simulink model "debug_conversion_debug"  (R2018b)
settings: configuration reference "Active" (kept outside this file)
settings Model: DataDictionary=mloc_debug_signal_conversion.sldd  Creator=ge34qer  LastModifiedBy=ge34qer

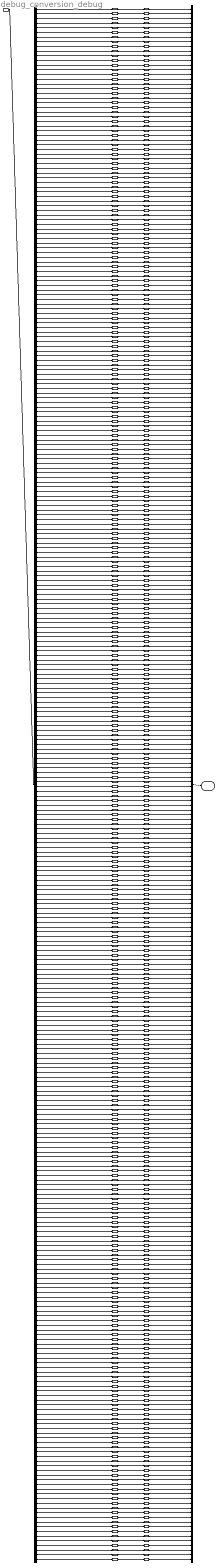
== system debug_conversion_debug ==
  debugIn : Inport  OutDataTypeStr=Bus: mvdc_vehicle_dynamics_control_debug
  BusOutput : BusSelector  OutputSignals=ErrorCode,mvdc_path_feedback_debug.Lat_FB_Sum_KappaReq_radpm,mvdc_path_feedback_debug.Lat_FB_Position,mvdc_path_feedback_debug.Lat_FB_Heading,mvdc_path_feedback_debug.Lat_LatPosError_m,mvdc_path_feedback_debug.Lat_LatPosError_DerAna_mps,mvdc_path_feedback_debug.Lat_LatPosError_DerNum_mps,mvdc_path_feedback_debug.Lat_LatPosError_DerDer_mps2,mvdc_path_feedback_debug.Lat_LatPosError_DerDerAna_mps2,mvdc_path_feedback_debug.Lat_LatPosError_DerDerNum_mps2,mvdc_path_feedback_debug.Lat_all_KappaReq_radpm,mvdc_path_matching_debug.PerformanceTrajOK_b,mvdc_path_matching_debug.EmergencyTrajOK_b,mvdc_path_matching_debug.PathPos.s_m,mvdc_path_matching_debug.PathPos.d_m,mvdc_path_matching_debug.PathPos.psi_rad,mvdc_path_matching_debug.ActualTrajPoint.LapCnt,mvdc_path_matching_debug.ActualTrajPoint.TrajCnt,mvdc_path_matching_debug.ActualTrajPoint.PointIdx,mvdc_path_matching_debug.ActualTrajPoint.s_loc_m,mvdc_path_matching_debug.ActualTrajPoint.s_glob_m,mvdc_path_matching_debug.ActualTrajPoint.x_m,mvdc_path_matching_debug.ActualTrajPoint.y_m,mvdc_path_matching_debug.ActualTrajPoint.psi_rad,mvdc_path_matching_debug.ActualTrajPoint.kappa_radpm,mvdc_path_matching_debug.ActualTrajPoint.v_mps,mvdc_path_matching_debug.ActualTrajPoint.ax_mps2,mvdc_path_matching_debug.ActualTrajPoint.banking_rad,mvdc_path_matching_debug.ActualTrajPoint.ax_lim_mps2,mvdc_path_matching_debug.ActualTrajPoint.ay_lim_mps2,mvdc_path_matching_debug.ActualTrajPoint.tube_r_m,mvdc_path_matching_debug.ActualTrajPoint.tube_l_m,mvdc_trajectory_driver_debug.ParkBrakeActive,mvdc_trajectory_driver_debug.DriverStatus,mvdc_trajectory_driver_debug.EnablePathMatching,mvdc_trajectory_driver_debug.EnableDriving,mvdc_trajectory_driver_debug.ControllerStatus,mvdc_trajectory_driver_debug.PathMatchingStatus,mvdc_trajectory_driver_debug.Strategy_Status,mvdc_trajectory_driver_debug.Trajectories_CommsStatus,mvdc_trajectory_driver_debug.Strategy_CommsStatus,mvdc_trajectory_driver_debug.tmpc_cnt,mvdc_trajectory_driver_perf.LapTime_s,mvdc_trajectory_driver_perf.e_lateral_m,mvdc_trajectory_driver_perf.eRMS_lateral_m,mvdc_trajectory_driver_perf.ePeak_lateral_m,mvdc_trajectory_driver_perf.e_heading_rad,mvdc_trajectory_driver_perf.eRMS_heading_rad,mvdc_trajectory_driver_perf.ePeak_heading_rad,mvdc_trajectory_driver_perf.e_v_mps,mvdc_trajectory_driver_perf.eRMS_v_mps,mvdc_trajectory_driver_perf.ePeak_v_mps,mvdc_trajectory_driver_perf.e_kappa_radpm,mvdc_trajectory_driver_perf.eRMS_kappa_radpm,mvdc_trajectory_driver_perf.ePeak_kappa_radpm,mvdc_trajectory_driver_perf.LongJerk_dax_mps3,mvdc_trajectory_driver_perf.LongJerkPeak_dax_mps3,mvdc_trajectory_driver_perf.LongJerkRMS_dax_mps3,mvdc_trajectory_driver_perf.LatJerk_day_mps3,mvdc_trajectory_driver_perf.LatJerkPeak_day_mps3,mvdc_trajectory_driver_perf.LatJerkRMS_day_mps3,mvdc_trajectory_driver_perf.SteeringRate_dDelta_radps,mvdc_trajectory_driver_perf.SteeringRatePeak_dDelta_radps,mvdc_trajectory_driver_perf.SteeringRateRMS_dDelta_radps,mvdc_trajectory_driver_perf.ForceRate_dF_Nps,mvdc_trajectory_driver_perf.ForceRatePeak_dF_Nps,mvdc_trajectory_driver_perf.ForceRateRMS_dF_Nps,mvdc_trajectory_driver_perf.LatConstViolations,mvdc_trajectory_driver_perf.TireConstViolations,mvdc_trajectory_driver_perf.TireUtilization,mvdc_trajectory_driver_perf.TireUtilization_c1,mvdc_trajectory_driver_perf.TireUtilization_c2,mvdc_curvvel_tracking_debug.Curv_TargetAy_mps2,mvdc_curvvel_tracking_debug.Curv_all_KappaReq_radpm,mvdc_curvvel_tracking_debug.Curv_FB_Dist_DeltaReq_rad,mvdc_curvvel_tracking_debug.Curv_FB_Diff_DeltaReq_rad,mvdc_curvvel_tracking_debug.Curv_FF_Kappa_DeltaReq_rad,mvdc_curvvel_tracking_debug.Curv_USComp_DeltaReq_rad,mvdc_curvvel_tracking_debug.Curv_CurvError_radpm,mvdc_curvvel_tracking_debug.Curv_TargetCurv_radpm,mvdc_curvvel_tracking_debug.Long_FB_Dist_FxReq_N,mvdc_curvvel_tracking_debug.Long_FF_Dist_FxReq_N,mvdc_curvvel_tracking_debug.Long_FB_VelDiff_FxReq_N,mvdc_curvvel_tracking_debug.Long_FF_Traj_FxReq_N,mvdc_curvvel_tracking_debug.Long_VelError_mps,mvdc_curvvel_tracking_debug.Long_TargetSpeed_mps,mvdc_curvvel_tracking_debug.Long_axTarget_mps2,mvdc_curvvel_tracking_debug.Req_Delta_rad,mvdc_curvvel_tracking_debug.Req_Fx_N,mvdc_curvvel_tracking_debug.ControlState,mvdc_curvvel_tracking_debug.EnableDriving,mvdc_curvvel_tracking_debug.EnableEmergency,mvdc_tmpc_fast_debug.LatAcc_bank_mps2,mvdc_tmpc_fast_debug.LatAcc_FB_Dist_rad,mvdc_tmpc_fast_debug.LatAcc_FB_ay_rad,mvdc_tmpc_fast_debug.LatAcc_FB_Delta_rad,mvdc_tmpc_fast_debug.LatAcc_FFss_rad,mvdc_tmpc_fast_debug.LatAcc_FFdyn_rad,mvdc_tmpc_fast_debug.LatAcc_Control_rad,mvdc_tmpc_fast_debug.LatAcc_Target_mps2,mvdc_tmpc_fast_debug.LatAcc_VirtualAccTarget_mps2,mvdc_tmpc_fast_debug.LatAcc_VirtualSteeringTarget_rad,mvdc_tmpc_fast_debug.LatAcc_FFLearned_rad,mvdc_tmpc_fast_debug.LatAcc_DiffToNeutralSteer_rad,mvdc_tmpc_fast_debug.LatAcc_FBStabilizer_rad,mvdc_tmpc_fast_debug.LongAcc_FB_N,mvdc_tmpc_fast_debug.LongAcc_FFax_N,mvdc_tmpc_fast_debug.LongAcc_FFdist_N,mvdc_tmpc_fast_debug.LongAcc_Control_N,mvdc_tmpc_fast_debug.LongAcc_Target_mps2,mvdc_tmpc_fast_debug.LongAcc_TargetFF_mps2,mvdc_tmpc_fast_debug.LongAcc_FFLearned_N,mvdc_tmpc_fast_debug.state_cost,mvdc_tmpc_fast_debug.input_cost,mvdc_tmpc_fast_debug.reg_cost,mvdc_tmpc_fast_debug.slack_cost,mvdc_tmpc_fast_debug.solver_iteration,mvdc_tmpc_fast_debug.solver_state,mvdc_tmpc_fast_debug.solver_runTime_s,mvdc_tmpc_fast_debug.solver_pri_res,mvdc_tmpc_fast_debug.solver_dua_res,mvdc_tmpc_fast_debug.tmpc_cnt,mvdc_tmpc_fast_debug.TireUtilizationTarget,mvdc_tmpc_fast_debug.ax_LearnedBound_mps2,mvdc_tmpc_fast_debug.ax_DataCoverage_perc,mvdc_tmpc_fast_debug.ax_Uncertainty_mps2,mvdc_tmpc_fast_debug.ay_LearnedBound_mps2,mvdc_tmpc_fast_debug.ay_DataCoverage_perc,mvdc_tmpc_fast_debug.ay_Uncertainty_mps2,mvdc_tmpc_fast_debug.dot_d_analytical_mps,mvdc_tmpc_fast_debug.dot_d_numerical_mps,mvdc_actuator_debug.steering_delta_target_rad,mvdc_actuator_debug.steering_delta_error_rad,mvdc_actuator_debug.steering_delta_FB_rad,mvdc_actuator_debug.steering_delta_FB_p_rad,mvdc_actuator_debug.steering_delta_FB_i_rad,mvdc_actuator_debug.steering_delta_FB_d_rad,mvdc_actuator_debug.steering_delta_FF_rad,mvdc_actuator_debug.RequestSteeringAngle_rad,mvdc_actuator_debug.RequestLongForce_N,mvdc_actuator_debug.TCCorrectiveForce_N,mvdc_actuator_debug.TCSlipDifference_perc,mvdc_actuator_debug.TCProportionalForce_N,mvdc_actuator_debug.TCIntegralForce_N,mvdc_actuator_debug.T_request_Nm,mvdc_actuator_debug.T_max_Nm,mvdc_actuator_debug.T_min_Nm,mvdc_actuator_debug.T_engine_Nm,mvdc_actuator_debug.p_Brake_bar,mvdc_actuator_debug.p_throttle_pos,mvdc_actuator_debug.gear,ExternalDebug.UnixTime_s,ExternalDebug.ExecutionTime_s,ExternalDebug.ControlTime_s,ExternalDebug.UpdateFrequency_Hz,ExternalDebug.LostHeartbeatTimeout_s,ExternalDebug.LostRaceControlTimeout_s,ExternalDebug.DiagSD,ExternalDebug.DiagMotec,ExternalDebug.DiagOther,mvdc_state_estimation_debug.StateEstimate.SE_Status,mvdc_state_estimation_debug.StateEstimate.SE_State,mvdc_state_estimation_debug.StateEstimate.Pos.x_m,mvdc_state_estimation_debug.StateEstimate.Pos.y_m,mvdc_state_estimation_debug.StateEstimate.Pos.psi_rad,mvdc_state_estimation_debug.StateEstimate.z_m,mvdc_state_estimation_debug.StateEstimate.PosAccuracy,mvdc_state_estimation_debug.StateEstimate.VelAccuracy,mvdc_state_estimation_debug.StateEstimate.dPsi_radps,mvdc_state_estimation_debug.StateEstimate.vx_mps,mvdc_state_estimation_debug.StateEstimate.vy_mps,mvdc_state_estimation_debug.StateEstimate.v_mps,mvdc_state_estimation_debug.StateEstimate.beta_rad,mvdc_state_estimation_debug.StateEstimate.ax_mps2,mvdc_state_estimation_debug.StateEstimate.ay_mps2,mvdc_state_estimation_debug.StateEstimate.valid_IMU_b,mvdc_state_estimation_debug.StateEstimate.psi_vel_rad,mvdc_state_estimation_debug.StateEstimate.kappa_radpm,mvdc_state_estimation_debug.StateEstimate.dBeta_radps,mvdc_state_estimation_debug.StateEstimate.ddPsi_radps2,mvdc_state_estimation_debug.StateEstimate.ax_vel_mps2,mvdc_state_estimation_debug.StateEstimate.ay_vel_mps2,mvdc_state_estimation_debug.StateEstimate.lambdaFL_perc,mvdc_state_estimation_debug.StateEstimate.lambdaFR_perc,mvdc_state_estimation_debug.StateEstimate.lambdaRL_perc,mvdc_state_estimation_debug.StateEstimate.lambdaRR_perc,mvdc_state_estimation_debug.StateEstimate.valid_Wheelspeeds_b,mvdc_state_estimation_debug.StateEstimate.alphaFL_rad,mvdc_state_estimation_debug.StateEstimate.alphaFR_rad,mvdc_state_estimation_debug.StateEstimate.alphaRL_rad,mvdc_state_estimation_debug.StateEstimate.alphaRR_rad,mvdc_state_estimation_debug.StateEstimate.DiffFRAlpha_rad,mvdc_state_estimation_debug.StateEstimate.DeltaWheel_rad,mvdc_state_estimation_debug.Residuals.res_xLoc1_m,mvdc_state_estimation_debug.Residuals.res_yLoc1_m,mvdc_state_estimation_debug.Residuals.res_psiLoc1_rad,mvdc_state_estimation_debug.Residuals.res_xLoc2_m,mvdc_state_estimation_debug.Residuals.res_yLoc2_m,mvdc_state_estimation_debug.Residuals.res_psiLoc2_rad,mvdc_state_estimation_debug.Residuals.res_xLoc3_m,mvdc_state_estimation_debug.Residuals.res_yLoc3_m,mvdc_state_estimation_debug.Residuals.res_psiLoc3_rad,mvdc_state_estimation_debug.Residuals.res_vxVel1_mps,mvdc_state_estimation_debug.Residuals.res_vyVel1_mps,mvdc_state_estimation_debug.Residuals.res_vxVel2_mps,mvdc_state_estimation_debug.Residuals.res_vyVel2_mps,mvdc_state_estimation_debug.Residuals.res_dPsi1_radps,mvdc_state_estimation_debug.Residuals.res_dPsi2_radps,mvdc_state_estimation_debug.Residuals.res_sLoc1_m,mvdc_state_estimation_debug.Residuals.res_dLoc1_m,mvdc_state_estimation_debug.Residuals.res_sLoc2_m,mvdc_state_estimation_debug.Residuals.res_dLoc2_m,mvdc_state_estimation_debug.Residuals.res_sLoc3_m,mvdc_state_estimation_debug.Residuals.res_dLoc3_m,mvdc_state_estimation_debug.Diagnosis.valid_Loc1_b,mvdc_state_estimation_debug.Diagnosis.valid_Loc2_b,mvdc_state_estimation_debug.Diagnosis.valid_Loc3_b,mvdc_state_estimation_debug.Diagnosis.valid_Vel1_b,mvdc_state_estimation_debug.Diagnosis.valid_Vel2_b,mvdc_state_estimation_debug.Diagnosis.valid_IMU1_b,mvdc_state_estimation_debug.Diagnosis.valid_IMU2_b,mvdc_state_estimation_debug.Diagnosis.fail_Loc1_b,mvdc_state_estimation_debug.Diagnosis.fail_Loc2_b,mvdc_state_estimation_debug.Diagnosis.fail_Loc3_b,mvdc_state_estimation_debug.Diagnosis.fail_Vel1_b,mvdc_state_estimation_debug.Diagnosis.fail_Vel2_b,mvdc_state_estimation_debug.Diagnosis.fail_IMU1_b,mvdc_state_estimation_debug.Diagnosis.fail_IMU2_b,mvdc_state_estimation_debug.Odom.Position.x_m,mvdc_state_estimation_debug.Odom.Position.y_m,mvdc_state_estimation_debug.Odom.Position.psi_rad,mvdc_state_estimation_debug.Odom.Valid_b,mloc_statemachine_debug.Hardware_Status,mloc_statemachine_debug.AIDriver_Status,mloc_statemachine_debug.ParkBrakeApplied_b,mloc_statemachine_debug.VehicleReady2Drive,mloc_statemachine_debug.StateEstimation_Status,mloc_statemachine_debug.VehicleSafeStandstill,mloc_statemachine_debug.Driver_Status,mloc_statemachine_debug.VehicleUnsafe,mloc_statemachine_debug.TUMVehicleState,mloc_statemachine_debug.EnableSensorFusion,mloc_statemachine_debug.EnableControlOutputs,mloc_statemachine_debug.EnableDriver,mloc_statemachine_debug.EnableHardEmergencyBrake,mloc_statemachine_debug.RequestControl,VehicleSensorData.s_DamperPotsFL_mm,VehicleSensorData.s_DamperPotsFR_mm,VehicleSensorData.s_DamperPotsRL_mm,VehicleSensorData.s_DamperPotsRR_mm,VehicleSensorData.p_TirePressureFL_bar,VehicleSensorData.p_TirePressureFR_bar,VehicleSensorData.p_TirePressureRL_bar,VehicleSensorData.p_TirePressureRR_bar,VehicleSensorData.T_TireFL_Celsius,VehicleSensorData.T_TireFR_Celsius,VehicleSensorData.T_TireRL_Celsius,VehicleSensorData.T_TireRR_Celsius,VehicleSensorData.BatteryVoltage_V,VehicleSensorData.Delta_Manual_rad,VehicleSensorData.Throttle_Manual_perc,VehicleSensorData.Brake_Manual_bar,VehicleSensorData.Gear_Manual,VehicleSensorData.T_CoolantTemp_Celsius,VehicleSensorData.T_TransmissionOilTemp_Celsius,VehicleSensorData.p_Fuel_kPa,VehicleSensorData.p_EngineOil_kPa,VehicleSensorData.Tz_Powertrain_Nm,VehicleSensorData.T_Engine_Nm,VehicleSensorData.GearEngaged,VehicleSensorData.omega_Engine_radps,VehicleSensorData.ThrottlePos_perc,VehicleSensorData.T_WheelFL_Nm,VehicleSensorData.T_WheelFR_Nm,VehicleSensorData.T_WheelRL_Nm,VehicleSensorData.T_WheelRR_Nm,VehicleSensorData.Delta_Wheel_rad,VehicleSensorData.p_BrakeF_bar,VehicleSensorData.p_BrakeR_bar,VehicleSensorData.omega_WheelFL_radps,VehicleSensorData.omega_WheelFR_radps,VehicleSensorData.omega_WheelRL_radps,VehicleSensorData.omega_WheelRR_radps,VehicleSensorData.valid_Wheelspeeds_b,VehicleSensorData.x_Loc1_m,VehicleSensorData.y_Loc1_m,VehicleSensorData.z_Loc1_m,VehicleSensorData.phi_RollAngleLoc1_rad,VehicleSensorData.theta_PitchAngleLoc1_rad,VehicleSensorData.psi_YawAngleLoc1_rad,VehicleSensorData.t_EstimateLoc1_s,VehicleSensorData.valid_Loc1_b,VehicleSensorData.accuracy_Loc1,VehicleSensorData.x_Loc2_m,VehicleSensorData.y_Loc2_m,VehicleSensorData.z_Loc2_m,VehicleSensorData.phi_RollAngleLoc2_rad,VehicleSensorData.theta_PitchAngleLoc2_rad,VehicleSensorData.psi_YawAngleLoc2_rad,VehicleSensorData.t_EstimateLoc2_s,VehicleSensorData.valid_Loc2_b,VehicleSensorData.accuracy_Loc2,VehicleSensorData.x_Loc3_m,VehicleSensorData.y_Loc3_m,VehicleSensorData.z_Loc3_m,VehicleSensorData.phi_RollAngleLoc3_rad,VehicleSensorData.theta_PitchAngleLoc3_rad,VehicleSensorData.psi_YawAngleLoc3_rad,VehicleSensorData.t_EstimateLoc3_s,VehicleSensorData.valid_Loc3_b,VehicleSensorData.accuracy_Loc3,VehicleSensorData.vx_CoGVel1_mps,VehicleSensorData.vy_CoGVel1_mps,VehicleSensorData.valid_Vel1_b,VehicleSensorData.vx_CoGVel2_mps,VehicleSensorData.vy_CoGVel2_mps,VehicleSensorData.valid_Vel2_b,VehicleSensorData.ax_CoGIMU1_mps2,VehicleSensorData.ay_CoGIMU1_mps2,VehicleSensorData.az_CoGIMU1_mps2,VehicleSensorData.dPhi_RollRateIMU1_radps,VehicleSensorData.dTheta_PitchRateIMU1_radps,VehicleSensorData.dPsi_YawRateIMU1_radps,VehicleSensorData.valid_IMU1_b,VehicleSensorData.ax_CoGIMU2_mps2,VehicleSensorData.ay_CoGIMU2_mps2,VehicleSensorData.az_CoGIMU2_mps2,VehicleSensorData.dPhi_RollRateIMU2_radps,VehicleSensorData.dTheta_PitchRateIMU2_radps,VehicleSensorData.dPsi_YawRateIMU2_radps,VehicleSensorData.valid_IMU2_b,Time_s
  Convert{1..332} (332 alike) : DataTypeConversion  OutDataTypeStr=double  SaturateOnIntegerOverflow=on  RndMeth=Zero
  Mux : Mux  Inputs=332
  debug_ErrorCode : SignalConversion  OverrideOpt=off
  debug_ExternalDebug_ControlTime_s : SignalConversion  OverrideOpt=off
  debug_ExternalDebug_DiagMotec : SignalConversion  OverrideOpt=off
  debug_ExternalDebug_DiagOther : SignalConversion  OverrideOpt=off
  debug_ExternalDebug_DiagSD : SignalConversion  OverrideOpt=off
  debug_ExternalDebug_ExecutionTime_s : SignalConversion  OverrideOpt=off
  debug_ExternalDebug_LostHeartbeatTimeout_s : SignalConversion  OverrideOpt=off
  debug_ExternalDebug_LostRaceControlTimeout_s : SignalConversion  OverrideOpt=off
  debug_ExternalDebug_UnixTime_s : SignalConversion  OverrideOpt=off
  debug_ExternalDebug_UpdateFrequency_Hz : SignalConversion  OverrideOpt=off
  debug_Time_s : SignalConversion  OverrideOpt=off
  debug_VehicleSensorData_BatteryVoltage_V : SignalConversion  OverrideOpt=off
  debug_VehicleSensorData_Brake_Manual_bar : SignalConversion  OverrideOpt=off
  debug_VehicleSensorData_Delta_Manual_rad : SignalConversion  OverrideOpt=off
  debug_VehicleSensorData_Delta_Wheel_rad : SignalConversion  OverrideOpt=off
  debug_VehicleSensorData_GearEngaged : SignalConversion  OverrideOpt=off
  debug_VehicleSensorData_Gear_Manual : SignalConversion  OverrideOpt=off
  debug_VehicleSensorData_T_CoolantTemp_Celsius : SignalConversion  OverrideOpt=off
  debug_VehicleSensorData_T_Engine_Nm : SignalConversion  OverrideOpt=off
  debug_VehicleSensorData_T_TireFL_Celsius : SignalConversion  OverrideOpt=off
  debug_VehicleSensorData_T_TireFR_Celsius : SignalConversion  OverrideOpt=off
  debug_VehicleSensorData_T_TireRL_Celsius : SignalConversion  OverrideOpt=off
  debug_VehicleSensorData_T_TireRR_Celsius : SignalConversion  OverrideOpt=off
  debug_VehicleSensorData_T_TransmissionOilTemp_Celsius : SignalConversion  OverrideOpt=off
  debug_VehicleSensorData_T_WheelFL_Nm : SignalConversion  OverrideOpt=off
  debug_VehicleSensorData_T_WheelFR_Nm : SignalConversion  OverrideOpt=off
  debug_VehicleSensorData_T_WheelRL_Nm : SignalConversion  OverrideOpt=off
  debug_VehicleSensorData_T_WheelRR_Nm : SignalConversion  OverrideOpt=off
  debug_VehicleSensorData_ThrottlePos_perc : SignalConversion  OverrideOpt=off
  debug_VehicleSensorData_Throttle_Manual_perc : SignalConversion  OverrideOpt=off
  debug_VehicleSensorData_Tz_Powertrain_Nm : SignalConversion  OverrideOpt=off
  debug_VehicleSensorData_accuracy_Loc1 : SignalConversion  OverrideOpt=off
  debug_VehicleSensorData_accuracy_Loc2 : SignalConversion  OverrideOpt=off
  debug_VehicleSensorData_accuracy_Loc3 : SignalConversion  OverrideOpt=off
  debug_VehicleSensorData_ax_CoGIMU1_mps2 : SignalConversion  OverrideOpt=off
  debug_VehicleSensorData_ax_CoGIMU2_mps2 : SignalConversion  OverrideOpt=off
  debug_VehicleSensorData_ay_CoGIMU1_mps2 : SignalConversion  OverrideOpt=off
  debug_VehicleSensorData_ay_CoGIMU2_mps2 : SignalConversion  OverrideOpt=off
  debug_VehicleSensorData_az_CoGIMU1_mps2 : SignalConversion  OverrideOpt=off
  debug_VehicleSensorData_az_CoGIMU2_mps2 : SignalConversion  OverrideOpt=off
  debug_VehicleSensorData_dPhi_RollRateIMU1_radps : SignalConversion  OverrideOpt=off
  debug_VehicleSensorData_dPhi_RollRateIMU2_radps : SignalConversion  OverrideOpt=off
  debug_VehicleSensorData_dPsi_YawRateIMU1_radps : SignalConversion  OverrideOpt=off
  debug_VehicleSensorData_dPsi_YawRateIMU2_radps : SignalConversion  OverrideOpt=off
  debug_VehicleSensorData_dTheta_PitchRateIMU1_radps : SignalConversion  OverrideOpt=off
  debug_VehicleSensorData_dTheta_PitchRateIMU2_radps : SignalConversion  OverrideOpt=off
  debug_VehicleSensorData_omega_Engine_radps : SignalConversion  OverrideOpt=off
  debug_VehicleSensorData_omega_WheelFL_radps : SignalConversion  OverrideOpt=off
  debug_VehicleSensorData_omega_WheelFR_radps : SignalConversion  OverrideOpt=off
  debug_VehicleSensorData_omega_WheelRL_radps : SignalConversion  OverrideOpt=off
  debug_VehicleSensorData_omega_WheelRR_radps : SignalConversion  OverrideOpt=off
  debug_VehicleSensorData_p_BrakeF_bar : SignalConversion  OverrideOpt=off
  debug_VehicleSensorData_p_BrakeR_bar : SignalConversion  OverrideOpt=off
  debug_VehicleSensorData_p_EngineOil_kPa : SignalConversion  OverrideOpt=off
  debug_VehicleSensorData_p_Fuel_kPa : SignalConversion  OverrideOpt=off
  debug_VehicleSensorData_p_TirePressureFL_bar : SignalConversion  OverrideOpt=off
  debug_VehicleSensorData_p_TirePressureFR_bar : SignalConversion  OverrideOpt=off
  debug_VehicleSensorData_p_TirePressureRL_bar : SignalConversion  OverrideOpt=off
  debug_VehicleSensorData_p_TirePressureRR_bar : SignalConversion  OverrideOpt=off
  debug_VehicleSensorData_phi_RollAngleLoc1_rad : SignalConversion  OverrideOpt=off
  debug_VehicleSensorData_phi_RollAngleLoc2_rad : SignalConversion  OverrideOpt=off
  debug_VehicleSensorData_phi_RollAngleLoc3_rad : SignalConversion  OverrideOpt=off
  debug_VehicleSensorData_psi_YawAngleLoc1_rad : SignalConversion  OverrideOpt=off
  debug_VehicleSensorData_psi_YawAngleLoc2_rad : SignalConversion  OverrideOpt=off
  debug_VehicleSensorData_psi_YawAngleLoc3_rad : SignalConversion  OverrideOpt=off
  debug_VehicleSensorData_s_DamperPotsFL_mm : SignalConversion  OverrideOpt=off
  debug_VehicleSensorData_s_DamperPotsFR_mm : SignalConversion  OverrideOpt=off
  debug_VehicleSensorData_s_DamperPotsRL_mm : SignalConversion  OverrideOpt=off
  debug_VehicleSensorData_s_DamperPotsRR_mm : SignalConversion  OverrideOpt=off
  debug_VehicleSensorData_t_EstimateLoc1_s : SignalConversion  OverrideOpt=off
  debug_VehicleSensorData_t_EstimateLoc2_s : SignalConversion  OverrideOpt=off
  debug_VehicleSensorData_t_EstimateLoc3_s : SignalConversion  OverrideOpt=off
  debug_VehicleSensorData_theta_PitchAngleLoc1_rad : SignalConversion  OverrideOpt=off
  debug_VehicleSensorData_theta_PitchAngleLoc2_rad : SignalConversion  OverrideOpt=off
  debug_VehicleSensorData_theta_PitchAngleLoc3_rad : SignalConversion  OverrideOpt=off
  debug_VehicleSensorData_valid_IMU1_b : SignalConversion  OverrideOpt=off
  debug_VehicleSensorData_valid_IMU2_b : SignalConversion  OverrideOpt=off
  debug_VehicleSensorData_valid_Loc1_b : SignalConversion  OverrideOpt=off
  debug_VehicleSensorData_valid_Loc2_b : SignalConversion  OverrideOpt=off
  debug_VehicleSensorData_valid_Loc3_b : SignalConversion  OverrideOpt=off
  debug_VehicleSensorData_valid_Vel1_b : SignalConversion  OverrideOpt=off
  debug_VehicleSensorData_valid_Vel2_b : SignalConversion  OverrideOpt=off
  debug_VehicleSensorData_valid_Wheelspeeds_b : SignalConversion  OverrideOpt=off
  debug_VehicleSensorData_vx_CoGVel1_mps : SignalConversion  OverrideOpt=off
  debug_VehicleSensorData_vx_CoGVel2_mps : SignalConversion  OverrideOpt=off
  debug_VehicleSensorData_vy_CoGVel1_mps : SignalConversion  OverrideOpt=off
  debug_VehicleSensorData_vy_CoGVel2_mps : SignalConversion  OverrideOpt=off
  debug_VehicleSensorData_x_Loc1_m : SignalConversion  OverrideOpt=off
  debug_VehicleSensorData_x_Loc2_m : SignalConversion  OverrideOpt=off
  debug_VehicleSensorData_x_Loc3_m : SignalConversion  OverrideOpt=off
  debug_VehicleSensorData_y_Loc1_m : SignalConversion  OverrideOpt=off
  debug_VehicleSensorData_y_Loc2_m : SignalConversion  OverrideOpt=off
  debug_VehicleSensorData_y_Loc3_m : SignalConversion  OverrideOpt=off
  debug_VehicleSensorData_z_Loc1_m : SignalConversion  OverrideOpt=off
  debug_VehicleSensorData_z_Loc2_m : SignalConversion  OverrideOpt=off
  debug_VehicleSensorData_z_Loc3_m : SignalConversion  OverrideOpt=off
  debug_mloc_statemachine_debug_AIDriver_Status : SignalConversion  OverrideOpt=off
  debug_mloc_statemachine_debug_Driver_Status : SignalConversion  OverrideOpt=off
  debug_mloc_statemachine_debug_EnableControlOutputs : SignalConversion  OverrideOpt=off
  debug_mloc_statemachine_debug_EnableDriver : SignalConversion  OverrideOpt=off
  debug_mloc_statemachine_debug_EnableHardEmergencyBrake : SignalConversion  OverrideOpt=off
  debug_mloc_statemachine_debug_EnableSensorFusion : SignalConversion  OverrideOpt=off
  debug_mloc_statemachine_debug_Hardware_Status : SignalConversion  OverrideOpt=off
  debug_mloc_statemachine_debug_ParkBrakeApplied_b : SignalConversion  OverrideOpt=off
  debug_mloc_statemachine_debug_RequestControl : SignalConversion  OverrideOpt=off
  debug_mloc_statemachine_debug_StateEstimation_Status : SignalConversion  OverrideOpt=off
  debug_mloc_statemachine_debug_TUMVehicleState : SignalConversion  OverrideOpt=off
  debug_mloc_statemachine_debug_VehicleReady2Drive : SignalConversion  OverrideOpt=off
  debug_mloc_statemachine_debug_VehicleSafeStandstill : SignalConversion  OverrideOpt=off
  debug_mloc_statemachine_debug_VehicleUnsafe : SignalConversion  OverrideOpt=off
  debug_mvdc_actuator_debug_RequestLongForce_N : SignalConversion  OverrideOpt=off
  debug_mvdc_actuator_debug_RequestSteeringAngle_rad : SignalConversion  OverrideOpt=off
  debug_mvdc_actuator_debug_TCCorrectiveForce_N : SignalConversion  OverrideOpt=off
  debug_mvdc_actuator_debug_TCIntegralForce_N : SignalConversion  OverrideOpt=off
  debug_mvdc_actuator_debug_TCProportionalForce_N : SignalConversion  OverrideOpt=off
  debug_mvdc_actuator_debug_TCSlipDifference_perc : SignalConversion  OverrideOpt=off
  debug_mvdc_actuator_debug_T_engine_Nm : SignalConversion  OverrideOpt=off
  debug_mvdc_actuator_debug_T_max_Nm : SignalConversion  OverrideOpt=off
  debug_mvdc_actuator_debug_T_min_Nm : SignalConversion  OverrideOpt=off
  debug_mvdc_actuator_debug_T_request_Nm : SignalConversion  OverrideOpt=off
  debug_mvdc_actuator_debug_gear : SignalConversion  OverrideOpt=off
  debug_mvdc_actuator_debug_p_Brake_bar : SignalConversion  OverrideOpt=off
  debug_mvdc_actuator_debug_p_throttle_pos : SignalConversion  OverrideOpt=off
  debug_mvdc_actuator_debug_steering_delta_FB_d_rad : SignalConversion  OverrideOpt=off
  debug_mvdc_actuator_debug_steering_delta_FB_i_rad : SignalConversion  OverrideOpt=off
  debug_mvdc_actuator_debug_steering_delta_FB_p_rad : SignalConversion  OverrideOpt=off
  debug_mvdc_actuator_debug_steering_delta_FB_rad : SignalConversion  OverrideOpt=off
  debug_mvdc_actuator_debug_steering_delta_FF_rad : SignalConversion  OverrideOpt=off
  debug_mvdc_actuator_debug_steering_delta_error_rad : SignalConversion  OverrideOpt=off
  debug_mvdc_actuator_debug_steering_delta_target_rad : SignalConversion  OverrideOpt=off
  debug_mvdc_curvvel_tracking_debug_ControlState : SignalConversion  OverrideOpt=off
  debug_mvdc_curvvel_tracking_debug_Curv_CurvError_radpm : SignalConversion  OverrideOpt=off
  debug_mvdc_curvvel_tracking_debug_Curv_FB_Diff_DeltaReq_rad : SignalConversion  OverrideOpt=off
  debug_mvdc_curvvel_tracking_debug_Curv_FB_Dist_DeltaReq_rad : SignalConversion  OverrideOpt=off
  debug_mvdc_curvvel_tracking_debug_Curv_FF_Kappa_DeltaReq_rad : SignalConversion  OverrideOpt=off
  debug_mvdc_curvvel_tracking_debug_Curv_TargetAy_mps2 : SignalConversion  OverrideOpt=off
  debug_mvdc_curvvel_tracking_debug_Curv_TargetCurv_radpm : SignalConversion  OverrideOpt=off
  debug_mvdc_curvvel_tracking_debug_Curv_USComp_DeltaReq_rad : SignalConversion  OverrideOpt=off
  debug_mvdc_curvvel_tracking_debug_Curv_all_KappaReq_radpm : SignalConversion  OverrideOpt=off
  debug_mvdc_curvvel_tracking_debug_EnableDriving : SignalConversion  OverrideOpt=off
  debug_mvdc_curvvel_tracking_debug_EnableEmergency : SignalConversion  OverrideOpt=off
  debug_mvdc_curvvel_tracking_debug_Long_FB_Dist_FxReq_N : SignalConversion  OverrideOpt=off
  debug_mvdc_curvvel_tracking_debug_Long_FB_VelDiff_FxReq_N : SignalConversion  OverrideOpt=off
  debug_mvdc_curvvel_tracking_debug_Long_FF_Dist_FxReq_N : SignalConversion  OverrideOpt=off
  debug_mvdc_curvvel_tracking_debug_Long_FF_Traj_FxReq_N : SignalConversion  OverrideOpt=off
  debug_mvdc_curvvel_tracking_debug_Long_TargetSpeed_mps : SignalConversion  OverrideOpt=off
  debug_mvdc_curvvel_tracking_debug_Long_VelError_mps : SignalConversion  OverrideOpt=off
  debug_mvdc_curvvel_tracking_debug_Long_axTarget_mps2 : SignalConversion  OverrideOpt=off
  debug_mvdc_curvvel_tracking_debug_Req_Delta_rad : SignalConversion  OverrideOpt=off
  debug_mvdc_curvvel_tracking_debug_Req_Fx_N : SignalConversion  OverrideOpt=off
  debug_mvdc_path_feedback_debug_Lat_FB_Heading : SignalConversion  OverrideOpt=off
  debug_mvdc_path_feedback_debug_Lat_FB_Position : SignalConversion  OverrideOpt=off
  debug_mvdc_path_feedback_debug_Lat_FB_Sum_KappaReq_radpm : SignalConversion  OverrideOpt=off
  debug_mvdc_path_feedback_debug_Lat_LatPosError_DerAna_mps : SignalConversion  OverrideOpt=off
  debug_mvdc_path_feedback_debug_Lat_LatPosError_DerDerAna_mps2 : SignalConversion  OverrideOpt=off
  debug_mvdc_path_feedback_debug_Lat_LatPosError_DerDerNum_mps2 : SignalConversion  OverrideOpt=off
  debug_mvdc_path_feedback_debug_Lat_LatPosError_DerDer_mps2 : SignalConversion  OverrideOpt=off
  debug_mvdc_path_feedback_debug_Lat_LatPosError_DerNum_mps : SignalConversion  OverrideOpt=off
  debug_mvdc_path_feedback_debug_Lat_LatPosError_m : SignalConversion  OverrideOpt=off
  debug_mvdc_path_feedback_debug_Lat_all_KappaReq_radpm : SignalConversion  OverrideOpt=off
  debug_mvdc_path_matching_debug_ActualTrajPoint_LapCnt : SignalConversion  OverrideOpt=off
  debug_mvdc_path_matching_debug_ActualTrajPoint_PointIdx : SignalConversion  OverrideOpt=off
  debug_mvdc_path_matching_debug_ActualTrajPoint_TrajCnt : SignalConversion  OverrideOpt=off
  debug_mvdc_path_matching_debug_ActualTrajPoint_ax_lim_mps2 : SignalConversion  OverrideOpt=off
  debug_mvdc_path_matching_debug_ActualTrajPoint_ax_mps2 : SignalConversion  OverrideOpt=off
  debug_mvdc_path_matching_debug_ActualTrajPoint_ay_lim_mps2 : SignalConversion  OverrideOpt=off
  debug_mvdc_path_matching_debug_ActualTrajPoint_banking_rad : SignalConversion  OverrideOpt=off
  debug_mvdc_path_matching_debug_ActualTrajPoint_kappa_radpm : SignalConversion  OverrideOpt=off
  debug_mvdc_path_matching_debug_ActualTrajPoint_psi_rad : SignalConversion  OverrideOpt=off
  debug_mvdc_path_matching_debug_ActualTrajPoint_s_glob_m : SignalConversion  OverrideOpt=off
  debug_mvdc_path_matching_debug_ActualTrajPoint_s_loc_m : SignalConversion  OverrideOpt=off
  debug_mvdc_path_matching_debug_ActualTrajPoint_tube_l_m : SignalConversion  OverrideOpt=off
  debug_mvdc_path_matching_debug_ActualTrajPoint_tube_r_m : SignalConversion  OverrideOpt=off
  debug_mvdc_path_matching_debug_ActualTrajPoint_v_mps : SignalConversion  OverrideOpt=off
  debug_mvdc_path_matching_debug_ActualTrajPoint_x_m : SignalConversion  OverrideOpt=off
  debug_mvdc_path_matching_debug_ActualTrajPoint_y_m : SignalConversion  OverrideOpt=off
  debug_mvdc_path_matching_debug_EmergencyTrajOK_b : SignalConversion  OverrideOpt=off
  debug_mvdc_path_matching_debug_PathPos_d_m : SignalConversion  OverrideOpt=off
  debug_mvdc_path_matching_debug_PathPos_psi_rad : SignalConversion  OverrideOpt=off
  debug_mvdc_path_matching_debug_PathPos_s_m : SignalConversion  OverrideOpt=off
  debug_mvdc_path_matching_debug_PerformanceTrajOK_b : SignalConversion  OverrideOpt=off
  debug_mvdc_state_estimation_debug_Diagnosis_fail_IMU1_b : SignalConversion  OverrideOpt=off
  debug_mvdc_state_estimation_debug_Diagnosis_fail_IMU2_b : SignalConversion  OverrideOpt=off
  debug_mvdc_state_estimation_debug_Diagnosis_fail_Loc1_b : SignalConversion  OverrideOpt=off
  debug_mvdc_state_estimation_debug_Diagnosis_fail_Loc2_b : SignalConversion  OverrideOpt=off
  debug_mvdc_state_estimation_debug_Diagnosis_fail_Loc3_b : SignalConversion  OverrideOpt=off
  debug_mvdc_state_estimation_debug_Diagnosis_fail_Vel1_b : SignalConversion  OverrideOpt=off
  debug_mvdc_state_estimation_debug_Diagnosis_fail_Vel2_b : SignalConversion  OverrideOpt=off
  debug_mvdc_state_estimation_debug_Diagnosis_valid_IMU1_b : SignalConversion  OverrideOpt=off
  debug_mvdc_state_estimation_debug_Diagnosis_valid_IMU2_b : SignalConversion  OverrideOpt=off
  debug_mvdc_state_estimation_debug_Diagnosis_valid_Loc1_b : SignalConversion  OverrideOpt=off
  debug_mvdc_state_estimation_debug_Diagnosis_valid_Loc2_b : SignalConversion  OverrideOpt=off
  debug_mvdc_state_estimation_debug_Diagnosis_valid_Loc3_b : SignalConversion  OverrideOpt=off
  debug_mvdc_state_estimation_debug_Diagnosis_valid_Vel1_b : SignalConversion  OverrideOpt=off
  debug_mvdc_state_estimation_debug_Diagnosis_valid_Vel2_b : SignalConversion  OverrideOpt=off
  debug_mvdc_state_estimation_debug_Odom_Position_psi_rad : SignalConversion  OverrideOpt=off
  debug_mvdc_state_estimation_debug_Odom_Position_x_m : SignalConversion  OverrideOpt=off
  debug_mvdc_state_estimation_debug_Odom_Position_y_m : SignalConversion  OverrideOpt=off
  debug_mvdc_state_estimation_debug_Odom_Valid_b : SignalConversion  OverrideOpt=off
  debug_mvdc_state_estimation_debug_Residuals_res_dLoc1_m : SignalConversion  OverrideOpt=off
  debug_mvdc_state_estimation_debug_Residuals_res_dLoc2_m : SignalConversion  OverrideOpt=off
  debug_mvdc_state_estimation_debug_Residuals_res_dLoc3_m : SignalConversion  OverrideOpt=off
  debug_mvdc_state_estimation_debug_Residuals_res_dPsi1_radps : SignalConversion  OverrideOpt=off
  debug_mvdc_state_estimation_debug_Residuals_res_dPsi2_radps : SignalConversion  OverrideOpt=off
  debug_mvdc_state_estimation_debug_Residuals_res_psiLoc1_rad : SignalConversion  OverrideOpt=off
  debug_mvdc_state_estimation_debug_Residuals_res_psiLoc2_rad : SignalConversion  OverrideOpt=off
  debug_mvdc_state_estimation_debug_Residuals_res_psiLoc3_rad : SignalConversion  OverrideOpt=off
  debug_mvdc_state_estimation_debug_Residuals_res_sLoc1_m : SignalConversion  OverrideOpt=off
  debug_mvdc_state_estimation_debug_Residuals_res_sLoc2_m : SignalConversion  OverrideOpt=off
  debug_mvdc_state_estimation_debug_Residuals_res_sLoc3_m : SignalConversion  OverrideOpt=off
  debug_mvdc_state_estimation_debug_Residuals_res_vxVel1_mps : SignalConversion  OverrideOpt=off
  debug_mvdc_state_estimation_debug_Residuals_res_vxVel2_mps : SignalConversion  OverrideOpt=off
  debug_mvdc_state_estimation_debug_Residuals_res_vyVel1_mps : SignalConversion  OverrideOpt=off
  debug_mvdc_state_estimation_debug_Residuals_res_vyVel2_mps : SignalConversion  OverrideOpt=off
  debug_mvdc_state_estimation_debug_Residuals_res_xLoc1_m : SignalConversion  OverrideOpt=off
  debug_mvdc_state_estimation_debug_Residuals_res_xLoc2_m : SignalConversion  OverrideOpt=off
  debug_mvdc_state_estimation_debug_Residuals_res_xLoc3_m : SignalConversion  OverrideOpt=off
  debug_mvdc_state_estimation_debug_Residuals_res_yLoc1_m : SignalConversion  OverrideOpt=off
  debug_mvdc_state_estimation_debug_Residuals_res_yLoc2_m : SignalConversion  OverrideOpt=off
  debug_mvdc_state_estimation_debug_Residuals_res_yLoc3_m : SignalConversion  OverrideOpt=off
  debug_mvdc_state_estimation_debug_StateEstimate_DeltaWheel_rad : SignalConversion  OverrideOpt=off
  debug_mvdc_state_estimation_debug_StateEstimate_DiffFRAlpha_rad : SignalConversion  OverrideOpt=off
  debug_mvdc_state_estimation_debug_StateEstimate_PosAccuracy : SignalConversion  OverrideOpt=off
  debug_mvdc_state_estimation_debug_StateEstimate_Pos_psi_rad : SignalConversion  OverrideOpt=off
  debug_mvdc_state_estimation_debug_StateEstimate_Pos_x_m : SignalConversion  OverrideOpt=off
  debug_mvdc_state_estimation_debug_StateEstimate_Pos_y_m : SignalConversion  OverrideOpt=off
  debug_mvdc_state_estimation_debug_StateEstimate_SE_State : SignalConversion  OverrideOpt=off
  debug_mvdc_state_estimation_debug_StateEstimate_SE_Status : SignalConversion  OverrideOpt=off
  debug_mvdc_state_estimation_debug_StateEstimate_VelAccuracy : SignalConversion  OverrideOpt=off
  debug_mvdc_state_estimation_debug_StateEstimate_alphaFL_rad : SignalConversion  OverrideOpt=off
  debug_mvdc_state_estimation_debug_StateEstimate_alphaFR_rad : SignalConversion  OverrideOpt=off
  debug_mvdc_state_estimation_debug_StateEstimate_alphaRL_rad : SignalConversion  OverrideOpt=off
  debug_mvdc_state_estimation_debug_StateEstimate_alphaRR_rad : SignalConversion  OverrideOpt=off
  debug_mvdc_state_estimation_debug_StateEstimate_ax_mps2 : SignalConversion  OverrideOpt=off
  debug_mvdc_state_estimation_debug_StateEstimate_ax_vel_mps2 : SignalConversion  OverrideOpt=off
  debug_mvdc_state_estimation_debug_StateEstimate_ay_mps2 : SignalConversion  OverrideOpt=off
  debug_mvdc_state_estimation_debug_StateEstimate_ay_vel_mps2 : SignalConversion  OverrideOpt=off
  debug_mvdc_state_estimation_debug_StateEstimate_beta_rad : SignalConversion  OverrideOpt=off
  debug_mvdc_state_estimation_debug_StateEstimate_dBeta_radps : SignalConversion  OverrideOpt=off
  debug_mvdc_state_estimation_debug_StateEstimate_dPsi_radps : SignalConversion  OverrideOpt=off
  debug_mvdc_state_estimation_debug_StateEstimate_ddPsi_radps2 : SignalConversion  OverrideOpt=off
  debug_mvdc_state_estimation_debug_StateEstimate_kappa_radpm : SignalConversion  OverrideOpt=off
  debug_mvdc_state_estimation_debug_StateEstimate_lambdaFL_perc : SignalConversion  OverrideOpt=off
  debug_mvdc_state_estimation_debug_StateEstimate_lambdaFR_perc : SignalConversion  OverrideOpt=off
  debug_mvdc_state_estimation_debug_StateEstimate_lambdaRL_perc : SignalConversion  OverrideOpt=off
  debug_mvdc_state_estimation_debug_StateEstimate_lambdaRR_perc : SignalConversion  OverrideOpt=off
  debug_mvdc_state_estimation_debug_StateEstimate_psi_vel_rad : SignalConversion  OverrideOpt=off
  debug_mvdc_state_estimation_debug_StateEstimate_v_mps : SignalConversion  OverrideOpt=off
  debug_mvdc_state_estimation_debug_StateEstimate_valid_IMU_b : SignalConversion  OverrideOpt=off
  debug_mvdc_state_estimation_debug_StateEstimate_valid_Wheelspeeds_b : SignalConversion  OverrideOpt=off
  debug_mvdc_state_estimation_debug_StateEstimate_vx_mps : SignalConversion  OverrideOpt=off
  debug_mvdc_state_estimation_debug_StateEstimate_vy_mps : SignalConversion  OverrideOpt=off
  debug_mvdc_state_estimation_debug_StateEstimate_z_m : SignalConversion  OverrideOpt=off
  debug_mvdc_tmpc_fast_debug_LatAcc_Control_rad : SignalConversion  OverrideOpt=off
  debug_mvdc_tmpc_fast_debug_LatAcc_DiffToNeutralSteer_rad : SignalConversion  OverrideOpt=off
  debug_mvdc_tmpc_fast_debug_LatAcc_FBStabilizer_rad : SignalConversion  OverrideOpt=off
  debug_mvdc_tmpc_fast_debug_LatAcc_FB_Delta_rad : SignalConversion  OverrideOpt=off
  debug_mvdc_tmpc_fast_debug_LatAcc_FB_Dist_rad : SignalConversion  OverrideOpt=off
  debug_mvdc_tmpc_fast_debug_LatAcc_FB_ay_rad : SignalConversion  OverrideOpt=off
  debug_mvdc_tmpc_fast_debug_LatAcc_FFLearned_rad : SignalConversion  OverrideOpt=off
  debug_mvdc_tmpc_fast_debug_LatAcc_FFdyn_rad : SignalConversion  OverrideOpt=off
  debug_mvdc_tmpc_fast_debug_LatAcc_FFss_rad : SignalConversion  OverrideOpt=off
  debug_mvdc_tmpc_fast_debug_LatAcc_Target_mps2 : SignalConversion  OverrideOpt=off
  debug_mvdc_tmpc_fast_debug_LatAcc_VirtualAccTarget_mps2 : SignalConversion  OverrideOpt=off
  debug_mvdc_tmpc_fast_debug_LatAcc_VirtualSteeringTarget_rad : SignalConversion  OverrideOpt=off
  debug_mvdc_tmpc_fast_debug_LatAcc_bank_mps2 : SignalConversion  OverrideOpt=off
  debug_mvdc_tmpc_fast_debug_LongAcc_Control_N : SignalConversion  OverrideOpt=off
  debug_mvdc_tmpc_fast_debug_LongAcc_FB_N : SignalConversion  OverrideOpt=off
  debug_mvdc_tmpc_fast_debug_LongAcc_FFLearned_N : SignalConversion  OverrideOpt=off
  debug_mvdc_tmpc_fast_debug_LongAcc_FFax_N : SignalConversion  OverrideOpt=off
  debug_mvdc_tmpc_fast_debug_LongAcc_FFdist_N : SignalConversion  OverrideOpt=off
  debug_mvdc_tmpc_fast_debug_LongAcc_TargetFF_mps2 : SignalConversion  OverrideOpt=off
  debug_mvdc_tmpc_fast_debug_LongAcc_Target_mps2 : SignalConversion  OverrideOpt=off
  debug_mvdc_tmpc_fast_debug_TireUtilizationTarget : SignalConversion  OverrideOpt=off
  debug_mvdc_tmpc_fast_debug_ax_DataCoverage_perc : SignalConversion  OverrideOpt=off
  debug_mvdc_tmpc_fast_debug_ax_LearnedBound_mps2 : SignalConversion  OverrideOpt=off
  debug_mvdc_tmpc_fast_debug_ax_Uncertainty_mps2 : SignalConversion  OverrideOpt=off
  debug_mvdc_tmpc_fast_debug_ay_DataCoverage_perc : SignalConversion  OverrideOpt=off
  debug_mvdc_tmpc_fast_debug_ay_LearnedBound_mps2 : SignalConversion  OverrideOpt=off
  debug_mvdc_tmpc_fast_debug_ay_Uncertainty_mps2 : SignalConversion  OverrideOpt=off
  debug_mvdc_tmpc_fast_debug_dot_d_analytical_mps : SignalConversion  OverrideOpt=off
  debug_mvdc_tmpc_fast_debug_dot_d_numerical_mps : SignalConversion  OverrideOpt=off
  debug_mvdc_tmpc_fast_debug_input_cost : SignalConversion  OverrideOpt=off
  debug_mvdc_tmpc_fast_debug_reg_cost : SignalConversion  OverrideOpt=off
  debug_mvdc_tmpc_fast_debug_slack_cost : SignalConversion  OverrideOpt=off
  debug_mvdc_tmpc_fast_debug_solver_dua_res : SignalConversion  OverrideOpt=off
  debug_mvdc_tmpc_fast_debug_solver_iteration : SignalConversion  OverrideOpt=off
  debug_mvdc_tmpc_fast_debug_solver_pri_res : SignalConversion  OverrideOpt=off
  debug_mvdc_tmpc_fast_debug_solver_runTime_s : SignalConversion  OverrideOpt=off
  debug_mvdc_tmpc_fast_debug_solver_state : SignalConversion  OverrideOpt=off
  debug_mvdc_tmpc_fast_debug_state_cost : SignalConversion  OverrideOpt=off
  debug_mvdc_tmpc_fast_debug_tmpc_cnt : SignalConversion  OverrideOpt=off
  debug_mvdc_trajectory_driver_debug_ControllerStatus : SignalConversion  OverrideOpt=off
  debug_mvdc_trajectory_driver_debug_DriverStatus : SignalConversion  OverrideOpt=off
  debug_mvdc_trajectory_driver_debug_EnableDriving : SignalConversion  OverrideOpt=off
  debug_mvdc_trajectory_driver_debug_EnablePathMatching : SignalConversion  OverrideOpt=off
  debug_mvdc_trajectory_driver_debug_ParkBrakeActive : SignalConversion  OverrideOpt=off
  debug_mvdc_trajectory_driver_debug_PathMatchingStatus : SignalConversion  OverrideOpt=off
  debug_mvdc_trajectory_driver_debug_Strategy_CommsStatus : SignalConversion  OverrideOpt=off
  debug_mvdc_trajectory_driver_debug_Strategy_Status : SignalConversion  OverrideOpt=off
  debug_mvdc_trajectory_driver_debug_Trajectories_CommsStatus : SignalConversion  OverrideOpt=off
  debug_mvdc_trajectory_driver_debug_tmpc_cnt : SignalConversion  OverrideOpt=off
  debug_mvdc_trajectory_driver_perf_ForceRatePeak_dF_Nps : SignalConversion  OverrideOpt=off
  debug_mvdc_trajectory_driver_perf_ForceRateRMS_dF_Nps : SignalConversion  OverrideOpt=off
  debug_mvdc_trajectory_driver_perf_ForceRate_dF_Nps : SignalConversion  OverrideOpt=off
  debug_mvdc_trajectory_driver_perf_LapTime_s : SignalConversion  OverrideOpt=off
  debug_mvdc_trajectory_driver_perf_LatConstViolations : SignalConversion  OverrideOpt=off
  debug_mvdc_trajectory_driver_perf_LatJerkPeak_day_mps3 : SignalConversion  OverrideOpt=off
  debug_mvdc_trajectory_driver_perf_LatJerkRMS_day_mps3 : SignalConversion  OverrideOpt=off
  debug_mvdc_trajectory_driver_perf_LatJerk_day_mps3 : SignalConversion  OverrideOpt=off
  debug_mvdc_trajectory_driver_perf_LongJerkPeak_dax_mps3 : SignalConversion  OverrideOpt=off
  debug_mvdc_trajectory_driver_perf_LongJerkRMS_dax_mps3 : SignalConversion  OverrideOpt=off
  debug_mvdc_trajectory_driver_perf_LongJerk_dax_mps3 : SignalConversion  OverrideOpt=off
  debug_mvdc_trajectory_driver_perf_SteeringRatePeak_dDelta_radps : SignalConversion  OverrideOpt=off
  debug_mvdc_trajectory_driver_perf_SteeringRateRMS_dDelta_radps : SignalConversion  OverrideOpt=off
  debug_mvdc_trajectory_driver_perf_SteeringRate_dDelta_radps : SignalConversion  OverrideOpt=off
  debug_mvdc_trajectory_driver_perf_TireConstViolations : SignalConversion  OverrideOpt=off
  debug_mvdc_trajectory_driver_perf_TireUtilization : SignalConversion  OverrideOpt=off
  debug_mvdc_trajectory_driver_perf_TireUtilization_c1 : SignalConversion  OverrideOpt=off
  debug_mvdc_trajectory_driver_perf_TireUtilization_c2 : SignalConversion  OverrideOpt=off
  debug_mvdc_trajectory_driver_perf_ePeak_heading_rad : SignalConversion  OverrideOpt=off
  debug_mvdc_trajectory_driver_perf_ePeak_kappa_radpm : SignalConversion  OverrideOpt=off
  debug_mvdc_trajectory_driver_perf_ePeak_lateral_m : SignalConversion  OverrideOpt=off
  debug_mvdc_trajectory_driver_perf_ePeak_v_mps : SignalConversion  OverrideOpt=off
  debug_mvdc_trajectory_driver_perf_eRMS_heading_rad : SignalConversion  OverrideOpt=off
  debug_mvdc_trajectory_driver_perf_eRMS_kappa_radpm : SignalConversion  OverrideOpt=off
  debug_mvdc_trajectory_driver_perf_eRMS_lateral_m : SignalConversion  OverrideOpt=off
  debug_mvdc_trajectory_driver_perf_eRMS_v_mps : SignalConversion  OverrideOpt=off
  debug_mvdc_trajectory_driver_perf_e_heading_rad : SignalConversion  OverrideOpt=off
  debug_mvdc_trajectory_driver_perf_e_kappa_radpm : SignalConversion  OverrideOpt=off
  debug_mvdc_trajectory_driver_perf_e_lateral_m : SignalConversion  OverrideOpt=off
  debug_mvdc_trajectory_driver_perf_e_v_mps : SignalConversion  OverrideOpt=off
  DebugOut : Outport
  wires:
  debugIn/1 -> BusOutput/1
  Convert1/1 -> debug_ErrorCode/1
  BusOutput/1 -> Convert1/1  "<ErrorCode>"
  debug_ErrorCode/1 -> Mux/1
  Convert2/1 -> debug_mvdc_path_feedback_debug_Lat_FB_Sum_KappaReq_radpm/1
  BusOutput/2 -> Convert2/1  "<Lat_FB_Sum_KappaReq_radpm>"
  debug_mvdc_path_feedback_debug_Lat_FB_Sum_KappaReq_radpm/1 -> Mux/2
  Convert3/1 -> debug_mvdc_path_feedback_debug_Lat_FB_Position/1
  BusOutput/3 -> Convert3/1  "<Lat_FB_Position>"
  debug_mvdc_path_feedback_debug_Lat_FB_Position/1 -> Mux/3
  Convert4/1 -> debug_mvdc_path_feedback_debug_Lat_FB_Heading/1
  BusOutput/4 -> Convert4/1  "<Lat_FB_Heading>"
  debug_mvdc_path_feedback_debug_Lat_FB_Heading/1 -> Mux/4
  Convert5/1 -> debug_mvdc_path_feedback_debug_Lat_LatPosError_m/1
  BusOutput/5 -> Convert5/1  "<Lat_LatPosError_m>"
  debug_mvdc_path_feedback_debug_Lat_LatPosError_m/1 -> Mux/5
  Convert6/1 -> debug_mvdc_path_feedback_debug_Lat_LatPosError_DerAna_mps/1
  BusOutput/6 -> Convert6/1  "<Lat_LatPosError_DerAna_mps>"
  debug_mvdc_path_feedback_debug_Lat_LatPosError_DerAna_mps/1 -> Mux/6
  Convert7/1 -> debug_mvdc_path_feedback_debug_Lat_LatPosError_DerNum_mps/1
  BusOutput/7 -> Convert7/1  "<Lat_LatPosError_DerNum_mps>"
  debug_mvdc_path_feedback_debug_Lat_LatPosError_DerNum_mps/1 -> Mux/7
  Convert8/1 -> debug_mvdc_path_feedback_debug_Lat_LatPosError_DerDer_mps2/1
  BusOutput/8 -> Convert8/1  "<Lat_LatPosError_DerDer_mps2>"
  debug_mvdc_path_feedback_debug_Lat_LatPosError_DerDer_mps2/1 -> Mux/8
  Convert9/1 -> debug_mvdc_path_feedback_debug_Lat_LatPosError_DerDerAna_mps2/1
  BusOutput/9 -> Convert9/1  "<Lat_LatPosError_DerDerAna_mps2>"
  debug_mvdc_path_feedback_debug_Lat_LatPosError_DerDerAna_mps2/1 -> Mux/9
  Convert10/1 -> debug_mvdc_path_feedback_debug_Lat_LatPosError_DerDerNum_mps2/1
  BusOutput/10 -> Convert10/1  "<Lat_LatPosError_DerDerNum_mps2>"
  debug_mvdc_path_feedback_debug_Lat_LatPosError_DerDerNum_mps2/1 -> Mux/10
  Convert11/1 -> debug_mvdc_path_feedback_debug_Lat_all_KappaReq_radpm/1
  BusOutput/11 -> Convert11/1  "<Lat_all_KappaReq_radpm>"
  debug_mvdc_path_feedback_debug_Lat_all_KappaReq_radpm/1 -> Mux/11
  Convert12/1 -> debug_mvdc_path_matching_debug_PerformanceTrajOK_b/1
  BusOutput/12 -> Convert12/1  "<PerformanceTrajOK_b>"
  debug_mvdc_path_matching_debug_PerformanceTrajOK_b/1 -> Mux/12
  Convert13/1 -> debug_mvdc_path_matching_debug_EmergencyTrajOK_b/1
  BusOutput/13 -> Convert13/1  "<EmergencyTrajOK_b>"
  debug_mvdc_path_matching_debug_EmergencyTrajOK_b/1 -> Mux/13
  Convert14/1 -> debug_mvdc_path_matching_debug_PathPos_s_m/1
  BusOutput/14 -> Convert14/1  "<s_m>"
  debug_mvdc_path_matching_debug_PathPos_s_m/1 -> Mux/14
  Convert15/1 -> debug_mvdc_path_matching_debug_PathPos_d_m/1
  BusOutput/15 -> Convert15/1  "<d_m>"
  debug_mvdc_path_matching_debug_PathPos_d_m/1 -> Mux/15
  Convert16/1 -> debug_mvdc_path_matching_debug_PathPos_psi_rad/1
  BusOutput/16 -> Convert16/1  "<psi_rad>"
  debug_mvdc_path_matching_debug_PathPos_psi_rad/1 -> Mux/16
  Convert17/1 -> debug_mvdc_path_matching_debug_ActualTrajPoint_LapCnt/1
  BusOutput/17 -> Convert17/1  "<LapCnt>"
  debug_mvdc_path_matching_debug_ActualTrajPoint_LapCnt/1 -> Mux/17
  Convert18/1 -> debug_mvdc_path_matching_debug_ActualTrajPoint_TrajCnt/1
  BusOutput/18 -> Convert18/1  "<TrajCnt>"
  debug_mvdc_path_matching_debug_ActualTrajPoint_TrajCnt/1 -> Mux/18
  Convert19/1 -> debug_mvdc_path_matching_debug_ActualTrajPoint_PointIdx/1
  BusOutput/19 -> Convert19/1  "<PointIdx>"
  debug_mvdc_path_matching_debug_ActualTrajPoint_PointIdx/1 -> Mux/19
  Convert20/1 -> debug_mvdc_path_matching_debug_ActualTrajPoint_s_loc_m/1
  BusOutput/20 -> Convert20/1  "<s_loc_m>"
  debug_mvdc_path_matching_debug_ActualTrajPoint_s_loc_m/1 -> Mux/20
  Convert21/1 -> debug_mvdc_path_matching_debug_ActualTrajPoint_s_glob_m/1
  BusOutput/21 -> Convert21/1  "<s_glob_m>"
  debug_mvdc_path_matching_debug_ActualTrajPoint_s_glob_m/1 -> Mux/21
  Convert22/1 -> debug_mvdc_path_matching_debug_ActualTrajPoint_x_m/1
  BusOutput/22 -> Convert22/1  "<x_m>"
  debug_mvdc_path_matching_debug_ActualTrajPoint_x_m/1 -> Mux/22
  Convert23/1 -> debug_mvdc_path_matching_debug_ActualTrajPoint_y_m/1
  BusOutput/23 -> Convert23/1  "<y_m>"
  debug_mvdc_path_matching_debug_ActualTrajPoint_y_m/1 -> Mux/23
  Convert24/1 -> debug_mvdc_path_matching_debug_ActualTrajPoint_psi_rad/1
  BusOutput/24 -> Convert24/1  "<psi_rad>"
  debug_mvdc_path_matching_debug_ActualTrajPoint_psi_rad/1 -> Mux/24
  Convert25/1 -> debug_mvdc_path_matching_debug_ActualTrajPoint_kappa_radpm/1
  BusOutput/25 -> Convert25/1  "<kappa_radpm>"
  debug_mvdc_path_matching_debug_ActualTrajPoint_kappa_radpm/1 -> Mux/25
  Convert26/1 -> debug_mvdc_path_matching_debug_ActualTrajPoint_v_mps/1
  BusOutput/26 -> Convert26/1  "<v_mps>"
  debug_mvdc_path_matching_debug_ActualTrajPoint_v_mps/1 -> Mux/26
  Convert27/1 -> debug_mvdc_path_matching_debug_ActualTrajPoint_ax_mps2/1
  BusOutput/27 -> Convert27/1  "<ax_mps2>"
  debug_mvdc_path_matching_debug_ActualTrajPoint_ax_mps2/1 -> Mux/27
  Convert28/1 -> debug_mvdc_path_matching_debug_ActualTrajPoint_banking_rad/1
  BusOutput/28 -> Convert28/1  "<banking_rad>"
  debug_mvdc_path_matching_debug_ActualTrajPoint_banking_rad/1 -> Mux/28
  Convert29/1 -> debug_mvdc_path_matching_debug_ActualTrajPoint_ax_lim_mps2/1
  BusOutput/29 -> Convert29/1  "<ax_lim_mps2>"
  debug_mvdc_path_matching_debug_ActualTrajPoint_ax_lim_mps2/1 -> Mux/29
  Convert30/1 -> debug_mvdc_path_matching_debug_ActualTrajPoint_ay_lim_mps2/1
  BusOutput/30 -> Convert30/1  "<ay_lim_mps2>"
  debug_mvdc_path_matching_debug_ActualTrajPoint_ay_lim_mps2/1 -> Mux/30
  Convert31/1 -> debug_mvdc_path_matching_debug_ActualTrajPoint_tube_r_m/1
  BusOutput/31 -> Convert31/1  "<tube_r_m>"
  debug_mvdc_path_matching_debug_ActualTrajPoint_tube_r_m/1 -> Mux/31
  Convert32/1 -> debug_mvdc_path_matching_debug_ActualTrajPoint_tube_l_m/1
  BusOutput/32 -> Convert32/1  "<tube_l_m>"
  debug_mvdc_path_matching_debug_ActualTrajPoint_tube_l_m/1 -> Mux/32
  Convert33/1 -> debug_mvdc_trajectory_driver_debug_ParkBrakeActive/1
  BusOutput/33 -> Convert33/1  "<ParkBrakeActive>"
  debug_mvdc_trajectory_driver_debug_ParkBrakeActive/1 -> Mux/33
  Convert34/1 -> debug_mvdc_trajectory_driver_debug_DriverStatus/1
  BusOutput/34 -> Convert34/1  "<DriverStatus>"
  debug_mvdc_trajectory_driver_debug_DriverStatus/1 -> Mux/34
  Convert35/1 -> debug_mvdc_trajectory_driver_debug_EnablePathMatching/1
  BusOutput/35 -> Convert35/1  "<EnablePathMatching>"
  debug_mvdc_trajectory_driver_debug_EnablePathMatching/1 -> Mux/35
  Convert36/1 -> debug_mvdc_trajectory_driver_debug_EnableDriving/1
  BusOutput/36 -> Convert36/1  "<EnableDriving>"
  debug_mvdc_trajectory_driver_debug_EnableDriving/1 -> Mux/36
  Convert37/1 -> debug_mvdc_trajectory_driver_debug_ControllerStatus/1
  BusOutput/37 -> Convert37/1  "<ControllerStatus>"
  debug_mvdc_trajectory_driver_debug_ControllerStatus/1 -> Mux/37
  Convert38/1 -> debug_mvdc_trajectory_driver_debug_PathMatchingStatus/1
  BusOutput/38 -> Convert38/1  "<PathMatchingStatus>"
  debug_mvdc_trajectory_driver_debug_PathMatchingStatus/1 -> Mux/38
  Convert39/1 -> debug_mvdc_trajectory_driver_debug_Strategy_Status/1
  BusOutput/39 -> Convert39/1  "<Strategy_Status>"
  debug_mvdc_trajectory_driver_debug_Strategy_Status/1 -> Mux/39
  Convert40/1 -> debug_mvdc_trajectory_driver_debug_Trajectories_CommsStatus/1
  BusOutput/40 -> Convert40/1  "<Trajectories_CommsStatus>"
  debug_mvdc_trajectory_driver_debug_Trajectories_CommsStatus/1 -> Mux/40
  Convert41/1 -> debug_mvdc_trajectory_driver_debug_Strategy_CommsStatus/1
  BusOutput/41 -> Convert41/1  "<Strategy_CommsStatus>"
  debug_mvdc_trajectory_driver_debug_Strategy_CommsStatus/1 -> Mux/41
  Convert42/1 -> debug_mvdc_trajectory_driver_debug_tmpc_cnt/1
  BusOutput/42 -> Convert42/1  "<tmpc_cnt>"
  debug_mvdc_trajectory_driver_debug_tmpc_cnt/1 -> Mux/42
  Convert43/1 -> debug_mvdc_trajectory_driver_perf_LapTime_s/1
  BusOutput/43 -> Convert43/1  "<LapTime_s>"
  debug_mvdc_trajectory_driver_perf_LapTime_s/1 -> Mux/43
  Convert44/1 -> debug_mvdc_trajectory_driver_perf_e_lateral_m/1
  BusOutput/44 -> Convert44/1  "<e_lateral_m>"
  debug_mvdc_trajectory_driver_perf_e_lateral_m/1 -> Mux/44
  Convert45/1 -> debug_mvdc_trajectory_driver_perf_eRMS_lateral_m/1
  BusOutput/45 -> Convert45/1  "<eRMS_lateral_m>"
  debug_mvdc_trajectory_driver_perf_eRMS_lateral_m/1 -> Mux/45
  Convert46/1 -> debug_mvdc_trajectory_driver_perf_ePeak_lateral_m/1
  BusOutput/46 -> Convert46/1  "<ePeak_lateral_m>"
  debug_mvdc_trajectory_driver_perf_ePeak_lateral_m/1 -> Mux/46
  Convert47/1 -> debug_mvdc_trajectory_driver_perf_e_heading_rad/1
  BusOutput/47 -> Convert47/1  "<e_heading_rad>"
  debug_mvdc_trajectory_driver_perf_e_heading_rad/1 -> Mux/47
  Convert48/1 -> debug_mvdc_trajectory_driver_perf_eRMS_heading_rad/1
  BusOutput/48 -> Convert48/1  "<eRMS_heading_rad>"
  debug_mvdc_trajectory_driver_perf_eRMS_heading_rad/1 -> Mux/48
  Convert49/1 -> debug_mvdc_trajectory_driver_perf_ePeak_heading_rad/1
  BusOutput/49 -> Convert49/1  "<ePeak_heading_rad>"
  debug_mvdc_trajectory_driver_perf_ePeak_heading_rad/1 -> Mux/49
  Convert50/1 -> debug_mvdc_trajectory_driver_perf_e_v_mps/1
  BusOutput/50 -> Convert50/1  "<e_v_mps>"
  debug_mvdc_trajectory_driver_perf_e_v_mps/1 -> Mux/50
  Convert51/1 -> debug_mvdc_trajectory_driver_perf_eRMS_v_mps/1
  BusOutput/51 -> Convert51/1  "<eRMS_v_mps>"
  debug_mvdc_trajectory_driver_perf_eRMS_v_mps/1 -> Mux/51
  Convert52/1 -> debug_mvdc_trajectory_driver_perf_ePeak_v_mps/1
  BusOutput/52 -> Convert52/1  "<ePeak_v_mps>"
  debug_mvdc_trajectory_driver_perf_ePeak_v_mps/1 -> Mux/52
  Convert53/1 -> debug_mvdc_trajectory_driver_perf_e_kappa_radpm/1
  BusOutput/53 -> Convert53/1  "<e_kappa_radpm>"
  debug_mvdc_trajectory_driver_perf_e_kappa_radpm/1 -> Mux/53
  Convert54/1 -> debug_mvdc_trajectory_driver_perf_eRMS_kappa_radpm/1
  BusOutput/54 -> Convert54/1  "<eRMS_kappa_radpm>"
  debug_mvdc_trajectory_driver_perf_eRMS_kappa_radpm/1 -> Mux/54
  Convert55/1 -> debug_mvdc_trajectory_driver_perf_ePeak_kappa_radpm/1
  BusOutput/55 -> Convert55/1  "<ePeak_kappa_radpm>"
  debug_mvdc_trajectory_driver_perf_ePeak_kappa_radpm/1 -> Mux/55
  Convert56/1 -> debug_mvdc_trajectory_driver_perf_LongJerk_dax_mps3/1
  BusOutput/56 -> Convert56/1  "<LongJerk_dax_mps3>"
  debug_mvdc_trajectory_driver_perf_LongJerk_dax_mps3/1 -> Mux/56
  Convert57/1 -> debug_mvdc_trajectory_driver_perf_LongJerkPeak_dax_mps3/1
  BusOutput/57 -> Convert57/1  "<LongJerkPeak_dax_mps3>"
  debug_mvdc_trajectory_driver_perf_LongJerkPeak_dax_mps3/1 -> Mux/57
  Convert58/1 -> debug_mvdc_trajectory_driver_perf_LongJerkRMS_dax_mps3/1
  BusOutput/58 -> Convert58/1  "<LongJerkRMS_dax_mps3>"
  debug_mvdc_trajectory_driver_perf_LongJerkRMS_dax_mps3/1 -> Mux/58
  Convert59/1 -> debug_mvdc_trajectory_driver_perf_LatJerk_day_mps3/1
  BusOutput/59 -> Convert59/1  "<LatJerk_day_mps3>"
  debug_mvdc_trajectory_driver_perf_LatJerk_day_mps3/1 -> Mux/59
  Convert60/1 -> debug_mvdc_trajectory_driver_perf_LatJerkPeak_day_mps3/1
  BusOutput/60 -> Convert60/1  "<LatJerkPeak_day_mps3>"
  debug_mvdc_trajectory_driver_perf_LatJerkPeak_day_mps3/1 -> Mux/60
  Convert61/1 -> debug_mvdc_trajectory_driver_perf_LatJerkRMS_day_mps3/1
  BusOutput/61 -> Convert61/1  "<LatJerkRMS_day_mps3>"
  debug_mvdc_trajectory_driver_perf_LatJerkRMS_day_mps3/1 -> Mux/61
  Convert62/1 -> debug_mvdc_trajectory_driver_perf_SteeringRate_dDelta_radps/1
  BusOutput/62 -> Convert62/1  "<SteeringRate_dDelta_radps>"
  debug_mvdc_trajectory_driver_perf_SteeringRate_dDelta_radps/1 -> Mux/62
  Convert63/1 -> debug_mvdc_trajectory_driver_perf_SteeringRatePeak_dDelta_radps/1
  BusOutput/63 -> Convert63/1  "<SteeringRatePeak_dDelta_radps>"
  debug_mvdc_trajectory_driver_perf_SteeringRatePeak_dDelta_radps/1 -> Mux/63
  Convert64/1 -> debug_mvdc_trajectory_driver_perf_SteeringRateRMS_dDelta_radps/1
  BusOutput/64 -> Convert64/1  "<SteeringRateRMS_dDelta_radps>"
  debug_mvdc_trajectory_driver_perf_SteeringRateRMS_dDelta_radps/1 -> Mux/64
  Convert65/1 -> debug_mvdc_trajectory_driver_perf_ForceRate_dF_Nps/1
  BusOutput/65 -> Convert65/1  "<ForceRate_dF_Nps>"
  debug_mvdc_trajectory_driver_perf_ForceRate_dF_Nps/1 -> Mux/65
  Convert66/1 -> debug_mvdc_trajectory_driver_perf_ForceRatePeak_dF_Nps/1
  BusOutput/66 -> Convert66/1  "<ForceRatePeak_dF_Nps>"
  debug_mvdc_trajectory_driver_perf_ForceRatePeak_dF_Nps/1 -> Mux/66
  Convert67/1 -> debug_mvdc_trajectory_driver_perf_ForceRateRMS_dF_Nps/1
  BusOutput/67 -> Convert67/1  "<ForceRateRMS_dF_Nps>"
  debug_mvdc_trajectory_driver_perf_ForceRateRMS_dF_Nps/1 -> Mux/67
  Convert68/1 -> debug_mvdc_trajectory_driver_perf_LatConstViolations/1
  BusOutput/68 -> Convert68/1  "<LatConstViolations>"
  debug_mvdc_trajectory_driver_perf_LatConstViolations/1 -> Mux/68
  Convert69/1 -> debug_mvdc_trajectory_driver_perf_TireConstViolations/1
  BusOutput/69 -> Convert69/1  "<TireConstViolations>"
  debug_mvdc_trajectory_driver_perf_TireConstViolations/1 -> Mux/69
  Convert70/1 -> debug_mvdc_trajectory_driver_perf_TireUtilization/1
  BusOutput/70 -> Convert70/1  "<TireUtilization>"
  debug_mvdc_trajectory_driver_perf_TireUtilization/1 -> Mux/70
  Convert71/1 -> debug_mvdc_trajectory_driver_perf_TireUtilization_c1/1
  BusOutput/71 -> Convert71/1  "<TireUtilization_c1>"
  debug_mvdc_trajectory_driver_perf_TireUtilization_c1/1 -> Mux/71
  Convert72/1 -> debug_mvdc_trajectory_driver_perf_TireUtilization_c2/1
  BusOutput/72 -> Convert72/1  "<TireUtilization_c2>"
  debug_mvdc_trajectory_driver_perf_TireUtilization_c2/1 -> Mux/72
  Convert73/1 -> debug_mvdc_curvvel_tracking_debug_Curv_TargetAy_mps2/1
  BusOutput/73 -> Convert73/1  "<Curv_TargetAy_mps2>"
  debug_mvdc_curvvel_tracking_debug_Curv_TargetAy_mps2/1 -> Mux/73
  Convert74/1 -> debug_mvdc_curvvel_tracking_debug_Curv_all_KappaReq_radpm/1
  BusOutput/74 -> Convert74/1  "<Curv_all_KappaReq_radpm>"
  debug_mvdc_curvvel_tracking_debug_Curv_all_KappaReq_radpm/1 -> Mux/74
  Convert75/1 -> debug_mvdc_curvvel_tracking_debug_Curv_FB_Dist_DeltaReq_rad/1
  BusOutput/75 -> Convert75/1  "<Curv_FB_Dist_DeltaReq_rad>"
  debug_mvdc_curvvel_tracking_debug_Curv_FB_Dist_DeltaReq_rad/1 -> Mux/75
  Convert76/1 -> debug_mvdc_curvvel_tracking_debug_Curv_FB_Diff_DeltaReq_rad/1
  BusOutput/76 -> Convert76/1  "<Curv_FB_Diff_DeltaReq_rad>"
  debug_mvdc_curvvel_tracking_debug_Curv_FB_Diff_DeltaReq_rad/1 -> Mux/76
  Convert77/1 -> debug_mvdc_curvvel_tracking_debug_Curv_FF_Kappa_DeltaReq_rad/1
  BusOutput/77 -> Convert77/1  "<Curv_FF_Kappa_DeltaReq_rad>"
  debug_mvdc_curvvel_tracking_debug_Curv_FF_Kappa_DeltaReq_rad/1 -> Mux/77
  Convert78/1 -> debug_mvdc_curvvel_tracking_debug_Curv_USComp_DeltaReq_rad/1
  BusOutput/78 -> Convert78/1  "<Curv_USComp_DeltaReq_rad>"
  debug_mvdc_curvvel_tracking_debug_Curv_USComp_DeltaReq_rad/1 -> Mux/78
  Convert79/1 -> debug_mvdc_curvvel_tracking_debug_Curv_CurvError_radpm/1
  BusOutput/79 -> Convert79/1  "<Curv_CurvError_radpm>"
  debug_mvdc_curvvel_tracking_debug_Curv_CurvError_radpm/1 -> Mux/79
  Convert80/1 -> debug_mvdc_curvvel_tracking_debug_Curv_TargetCurv_radpm/1
  BusOutput/80 -> Convert80/1  "<Curv_TargetCurv_radpm>"
  debug_mvdc_curvvel_tracking_debug_Curv_TargetCurv_radpm/1 -> Mux/80
  Convert81/1 -> debug_mvdc_curvvel_tracking_debug_Long_FB_Dist_FxReq_N/1
  BusOutput/81 -> Convert81/1  "<Long_FB_Dist_FxReq_N>"
  debug_mvdc_curvvel_tracking_debug_Long_FB_Dist_FxReq_N/1 -> Mux/81
  Convert82/1 -> debug_mvdc_curvvel_tracking_debug_Long_FF_Dist_FxReq_N/1
  BusOutput/82 -> Convert82/1  "<Long_FF_Dist_FxReq_N>"
  debug_mvdc_curvvel_tracking_debug_Long_FF_Dist_FxReq_N/1 -> Mux/82
  Convert83/1 -> debug_mvdc_curvvel_tracking_debug_Long_FB_VelDiff_FxReq_N/1
  BusOutput/83 -> Convert83/1  "<Long_FB_VelDiff_FxReq_N>"
  debug_mvdc_curvvel_tracking_debug_Long_FB_VelDiff_FxReq_N/1 -> Mux/83
  Convert84/1 -> debug_mvdc_curvvel_tracking_debug_Long_FF_Traj_FxReq_N/1
  BusOutput/84 -> Convert84/1  "<Long_FF_Traj_FxReq_N>"
  debug_mvdc_curvvel_tracking_debug_Long_FF_Traj_FxReq_N/1 -> Mux/84
  Convert85/1 -> debug_mvdc_curvvel_tracking_debug_Long_VelError_mps/1
  BusOutput/85 -> Convert85/1  "<Long_VelError_mps>"
  debug_mvdc_curvvel_tracking_debug_Long_VelError_mps/1 -> Mux/85
  Convert86/1 -> debug_mvdc_curvvel_tracking_debug_Long_TargetSpeed_mps/1
  BusOutput/86 -> Convert86/1  "<Long_TargetSpeed_mps>"
  debug_mvdc_curvvel_tracking_debug_Long_TargetSpeed_mps/1 -> Mux/86
  Convert87/1 -> debug_mvdc_curvvel_tracking_debug_Long_axTarget_mps2/1
  BusOutput/87 -> Convert87/1  "<Long_axTarget_mps2>"
  debug_mvdc_curvvel_tracking_debug_Long_axTarget_mps2/1 -> Mux/87
  Convert88/1 -> debug_mvdc_curvvel_tracking_debug_Req_Delta_rad/1
  BusOutput/88 -> Convert88/1  "<Req_Delta_rad>"
  debug_mvdc_curvvel_tracking_debug_Req_Delta_rad/1 -> Mux/88
  Convert89/1 -> debug_mvdc_curvvel_tracking_debug_Req_Fx_N/1
  BusOutput/89 -> Convert89/1  "<Req_Fx_N>"
  debug_mvdc_curvvel_tracking_debug_Req_Fx_N/1 -> Mux/89
  Convert90/1 -> debug_mvdc_curvvel_tracking_debug_ControlState/1
  BusOutput/90 -> Convert90/1  "<ControlState>"
  debug_mvdc_curvvel_tracking_debug_ControlState/1 -> Mux/90
  Convert91/1 -> debug_mvdc_curvvel_tracking_debug_EnableDriving/1
  BusOutput/91 -> Convert91/1  "<EnableDriving>"
  debug_mvdc_curvvel_tracking_debug_EnableDriving/1 -> Mux/91
  Convert92/1 -> debug_mvdc_curvvel_tracking_debug_EnableEmergency/1
  BusOutput/92 -> Convert92/1  "<EnableEmergency>"
  debug_mvdc_curvvel_tracking_debug_EnableEmergency/1 -> Mux/92
  Convert93/1 -> debug_mvdc_tmpc_fast_debug_LatAcc_bank_mps2/1
  BusOutput/93 -> Convert93/1  "<LatAcc_bank_mps2>"
  debug_mvdc_tmpc_fast_debug_LatAcc_bank_mps2/1 -> Mux/93
  Convert94/1 -> debug_mvdc_tmpc_fast_debug_LatAcc_FB_Dist_rad/1
  BusOutput/94 -> Convert94/1  "<LatAcc_FB_Dist_rad>"
  debug_mvdc_tmpc_fast_debug_LatAcc_FB_Dist_rad/1 -> Mux/94
  Convert95/1 -> debug_mvdc_tmpc_fast_debug_LatAcc_FB_ay_rad/1
  BusOutput/95 -> Convert95/1  "<LatAcc_FB_ay_rad>"
  debug_mvdc_tmpc_fast_debug_LatAcc_FB_ay_rad/1 -> Mux/95
  Convert96/1 -> debug_mvdc_tmpc_fast_debug_LatAcc_FB_Delta_rad/1
  BusOutput/96 -> Convert96/1  "<LatAcc_FB_Delta_rad>"
  debug_mvdc_tmpc_fast_debug_LatAcc_FB_Delta_rad/1 -> Mux/96
  Convert97/1 -> debug_mvdc_tmpc_fast_debug_LatAcc_FFss_rad/1
  BusOutput/97 -> Convert97/1  "<LatAcc_FFss_rad>"
  debug_mvdc_tmpc_fast_debug_LatAcc_FFss_rad/1 -> Mux/97
  Convert98/1 -> debug_mvdc_tmpc_fast_debug_LatAcc_FFdyn_rad/1
  BusOutput/98 -> Convert98/1  "<LatAcc_FFdyn_rad>"
  debug_mvdc_tmpc_fast_debug_LatAcc_FFdyn_rad/1 -> Mux/98
  Convert99/1 -> debug_mvdc_tmpc_fast_debug_LatAcc_Control_rad/1
  BusOutput/99 -> Convert99/1  "<LatAcc_Control_rad>"
  debug_mvdc_tmpc_fast_debug_LatAcc_Control_rad/1 -> Mux/99
  Convert100/1 -> debug_mvdc_tmpc_fast_debug_LatAcc_Target_mps2/1
  BusOutput/100 -> Convert100/1  "<LatAcc_Target_mps2>"
  debug_mvdc_tmpc_fast_debug_LatAcc_Target_mps2/1 -> Mux/100
  Convert101/1 -> debug_mvdc_tmpc_fast_debug_LatAcc_VirtualAccTarget_mps2/1
  BusOutput/101 -> Convert101/1  "<LatAcc_VirtualAccTarget_mps2>"
  debug_mvdc_tmpc_fast_debug_LatAcc_VirtualAccTarget_mps2/1 -> Mux/101
  Convert102/1 -> debug_mvdc_tmpc_fast_debug_LatAcc_VirtualSteeringTarget_rad/1
  BusOutput/102 -> Convert102/1  "<LatAcc_VirtualSteeringTarget_rad>"
  debug_mvdc_tmpc_fast_debug_LatAcc_VirtualSteeringTarget_rad/1 -> Mux/102
  Convert103/1 -> debug_mvdc_tmpc_fast_debug_LatAcc_FFLearned_rad/1
  BusOutput/103 -> Convert103/1  "<LatAcc_FFLearned_rad>"
  debug_mvdc_tmpc_fast_debug_LatAcc_FFLearned_rad/1 -> Mux/103
  Convert104/1 -> debug_mvdc_tmpc_fast_debug_LatAcc_DiffToNeutralSteer_rad/1
  BusOutput/104 -> Convert104/1  "<LatAcc_DiffToNeutralSteer_rad>"
  debug_mvdc_tmpc_fast_debug_LatAcc_DiffToNeutralSteer_rad/1 -> Mux/104
  Convert105/1 -> debug_mvdc_tmpc_fast_debug_LatAcc_FBStabilizer_rad/1
  BusOutput/105 -> Convert105/1  "<LatAcc_FBStabilizer_rad>"
  debug_mvdc_tmpc_fast_debug_LatAcc_FBStabilizer_rad/1 -> Mux/105
  Convert106/1 -> debug_mvdc_tmpc_fast_debug_LongAcc_FB_N/1
  BusOutput/106 -> Convert106/1  "<LongAcc_FB_N>"
  debug_mvdc_tmpc_fast_debug_LongAcc_FB_N/1 -> Mux/106
  Convert107/1 -> debug_mvdc_tmpc_fast_debug_LongAcc_FFax_N/1
  BusOutput/107 -> Convert107/1  "<LongAcc_FFax_N>"
  debug_mvdc_tmpc_fast_debug_LongAcc_FFax_N/1 -> Mux/107
  Convert108/1 -> debug_mvdc_tmpc_fast_debug_LongAcc_FFdist_N/1
  BusOutput/108 -> Convert108/1  "<LongAcc_FFdist_N>"
  debug_mvdc_tmpc_fast_debug_LongAcc_FFdist_N/1 -> Mux/108
  Convert109/1 -> debug_mvdc_tmpc_fast_debug_LongAcc_Control_N/1
  BusOutput/109 -> Convert109/1  "<LongAcc_Control_N>"
  debug_mvdc_tmpc_fast_debug_LongAcc_Control_N/1 -> Mux/109
  Convert110/1 -> debug_mvdc_tmpc_fast_debug_LongAcc_Target_mps2/1
  BusOutput/110 -> Convert110/1  "<LongAcc_Target_mps2>"
  debug_mvdc_tmpc_fast_debug_LongAcc_Target_mps2/1 -> Mux/110
  Convert111/1 -> debug_mvdc_tmpc_fast_debug_LongAcc_TargetFF_mps2/1
  BusOutput/111 -> Convert111/1  "<LongAcc_TargetFF_mps2>"
  debug_mvdc_tmpc_fast_debug_LongAcc_TargetFF_mps2/1 -> Mux/111
  Convert112/1 -> debug_mvdc_tmpc_fast_debug_LongAcc_FFLearned_N/1
  BusOutput/112 -> Convert112/1  "<LongAcc_FFLearned_N>"
  debug_mvdc_tmpc_fast_debug_LongAcc_FFLearned_N/1 -> Mux/112
  Convert113/1 -> debug_mvdc_tmpc_fast_debug_state_cost/1
  BusOutput/113 -> Convert113/1  "<state_cost>"
  debug_mvdc_tmpc_fast_debug_state_cost/1 -> Mux/113
  Convert114/1 -> debug_mvdc_tmpc_fast_debug_input_cost/1
  BusOutput/114 -> Convert114/1  "<input_cost>"
  debug_mvdc_tmpc_fast_debug_input_cost/1 -> Mux/114
  Convert115/1 -> debug_mvdc_tmpc_fast_debug_reg_cost/1
  BusOutput/115 -> Convert115/1  "<reg_cost>"
  debug_mvdc_tmpc_fast_debug_reg_cost/1 -> Mux/115
  Convert116/1 -> debug_mvdc_tmpc_fast_debug_slack_cost/1
  BusOutput/116 -> Convert116/1  "<slack_cost>"
  debug_mvdc_tmpc_fast_debug_slack_cost/1 -> Mux/116
  Convert117/1 -> debug_mvdc_tmpc_fast_debug_solver_iteration/1
  BusOutput/117 -> Convert117/1  "<solver_iteration>"
  debug_mvdc_tmpc_fast_debug_solver_iteration/1 -> Mux/117
  Convert118/1 -> debug_mvdc_tmpc_fast_debug_solver_state/1
  BusOutput/118 -> Convert118/1  "<solver_state>"
  debug_mvdc_tmpc_fast_debug_solver_state/1 -> Mux/118
  Convert119/1 -> debug_mvdc_tmpc_fast_debug_solver_runTime_s/1
  BusOutput/119 -> Convert119/1  "<solver_runTime_s>"
  debug_mvdc_tmpc_fast_debug_solver_runTime_s/1 -> Mux/119
  Convert120/1 -> debug_mvdc_tmpc_fast_debug_solver_pri_res/1
  BusOutput/120 -> Convert120/1  "<solver_pri_res>"
  debug_mvdc_tmpc_fast_debug_solver_pri_res/1 -> Mux/120
  Convert121/1 -> debug_mvdc_tmpc_fast_debug_solver_dua_res/1
  BusOutput/121 -> Convert121/1  "<solver_dua_res>"
  debug_mvdc_tmpc_fast_debug_solver_dua_res/1 -> Mux/121
  Convert122/1 -> debug_mvdc_tmpc_fast_debug_tmpc_cnt/1
  BusOutput/122 -> Convert122/1  "<tmpc_cnt>"
  debug_mvdc_tmpc_fast_debug_tmpc_cnt/1 -> Mux/122
  Convert123/1 -> debug_mvdc_tmpc_fast_debug_TireUtilizationTarget/1
  BusOutput/123 -> Convert123/1  "<TireUtilizationTarget>"
  debug_mvdc_tmpc_fast_debug_TireUtilizationTarget/1 -> Mux/123
  Convert124/1 -> debug_mvdc_tmpc_fast_debug_ax_LearnedBound_mps2/1
  BusOutput/124 -> Convert124/1  "<ax_LearnedBound_mps2>"
  debug_mvdc_tmpc_fast_debug_ax_LearnedBound_mps2/1 -> Mux/124
  Convert125/1 -> debug_mvdc_tmpc_fast_debug_ax_DataCoverage_perc/1
  BusOutput/125 -> Convert125/1  "<ax_DataCoverage_perc>"
  debug_mvdc_tmpc_fast_debug_ax_DataCoverage_perc/1 -> Mux/125
  Convert126/1 -> debug_mvdc_tmpc_fast_debug_ax_Uncertainty_mps2/1
  BusOutput/126 -> Convert126/1  "<ax_Uncertainty_mps2>"
  debug_mvdc_tmpc_fast_debug_ax_Uncertainty_mps2/1 -> Mux/126
  Convert127/1 -> debug_mvdc_tmpc_fast_debug_ay_LearnedBound_mps2/1
  BusOutput/127 -> Convert127/1  "<ay_LearnedBound_mps2>"
  debug_mvdc_tmpc_fast_debug_ay_LearnedBound_mps2/1 -> Mux/127
  Convert128/1 -> debug_mvdc_tmpc_fast_debug_ay_DataCoverage_perc/1
  BusOutput/128 -> Convert128/1  "<ay_DataCoverage_perc>"
  debug_mvdc_tmpc_fast_debug_ay_DataCoverage_perc/1 -> Mux/128
  Convert129/1 -> debug_mvdc_tmpc_fast_debug_ay_Uncertainty_mps2/1
  BusOutput/129 -> Convert129/1  "<ay_Uncertainty_mps2>"
  debug_mvdc_tmpc_fast_debug_ay_Uncertainty_mps2/1 -> Mux/129
  Convert130/1 -> debug_mvdc_tmpc_fast_debug_dot_d_analytical_mps/1
  BusOutput/130 -> Convert130/1  "<dot_d_analytical_mps>"
  debug_mvdc_tmpc_fast_debug_dot_d_analytical_mps/1 -> Mux/130
  Convert131/1 -> debug_mvdc_tmpc_fast_debug_dot_d_numerical_mps/1
  BusOutput/131 -> Convert131/1  "<dot_d_numerical_mps>"
  debug_mvdc_tmpc_fast_debug_dot_d_numerical_mps/1 -> Mux/131
  Convert132/1 -> debug_mvdc_actuator_debug_steering_delta_target_rad/1
  BusOutput/132 -> Convert132/1  "<steering_delta_target_rad>"
  debug_mvdc_actuator_debug_steering_delta_target_rad/1 -> Mux/132
  Convert133/1 -> debug_mvdc_actuator_debug_steering_delta_error_rad/1
  BusOutput/133 -> Convert133/1  "<steering_delta_error_rad>"
  debug_mvdc_actuator_debug_steering_delta_error_rad/1 -> Mux/133
  Convert134/1 -> debug_mvdc_actuator_debug_steering_delta_FB_rad/1
  BusOutput/134 -> Convert134/1  "<steering_delta_FB_rad>"
  debug_mvdc_actuator_debug_steering_delta_FB_rad/1 -> Mux/134
  Convert135/1 -> debug_mvdc_actuator_debug_steering_delta_FB_p_rad/1
  BusOutput/135 -> Convert135/1  "<steering_delta_FB_p_rad>"
  debug_mvdc_actuator_debug_steering_delta_FB_p_rad/1 -> Mux/135
  Convert136/1 -> debug_mvdc_actuator_debug_steering_delta_FB_i_rad/1
  BusOutput/136 -> Convert136/1  "<steering_delta_FB_i_rad>"
  debug_mvdc_actuator_debug_steering_delta_FB_i_rad/1 -> Mux/136
  Convert137/1 -> debug_mvdc_actuator_debug_steering_delta_FB_d_rad/1
  BusOutput/137 -> Convert137/1  "<steering_delta_FB_d_rad>"
  debug_mvdc_actuator_debug_steering_delta_FB_d_rad/1 -> Mux/137
  Convert138/1 -> debug_mvdc_actuator_debug_steering_delta_FF_rad/1
  BusOutput/138 -> Convert138/1  "<steering_delta_FF_rad>"
  debug_mvdc_actuator_debug_steering_delta_FF_rad/1 -> Mux/138
  Convert139/1 -> debug_mvdc_actuator_debug_RequestSteeringAngle_rad/1
  BusOutput/139 -> Convert139/1  "<RequestSteeringAngle_rad>"
  debug_mvdc_actuator_debug_RequestSteeringAngle_rad/1 -> Mux/139
  Convert140/1 -> debug_mvdc_actuator_debug_RequestLongForce_N/1
  BusOutput/140 -> Convert140/1  "<RequestLongForce_N>"
  debug_mvdc_actuator_debug_RequestLongForce_N/1 -> Mux/140
  Convert141/1 -> debug_mvdc_actuator_debug_TCCorrectiveForce_N/1
  BusOutput/141 -> Convert141/1  "<TCCorrectiveForce_N>"
  debug_mvdc_actuator_debug_TCCorrectiveForce_N/1 -> Mux/141
  Convert142/1 -> debug_mvdc_actuator_debug_TCSlipDifference_perc/1
  BusOutput/142 -> Convert142/1  "<TCSlipDifference_perc>"
  debug_mvdc_actuator_debug_TCSlipDifference_perc/1 -> Mux/142
  Convert143/1 -> debug_mvdc_actuator_debug_TCProportionalForce_N/1
  BusOutput/143 -> Convert143/1  "<TCProportionalForce_N>"
  debug_mvdc_actuator_debug_TCProportionalForce_N/1 -> Mux/143
  Convert144/1 -> debug_mvdc_actuator_debug_TCIntegralForce_N/1
  BusOutput/144 -> Convert144/1  "<TCIntegralForce_N>"
  debug_mvdc_actuator_debug_TCIntegralForce_N/1 -> Mux/144
  Convert145/1 -> debug_mvdc_actuator_debug_T_request_Nm/1
  BusOutput/145 -> Convert145/1  "<T_request_Nm>"
  debug_mvdc_actuator_debug_T_request_Nm/1 -> Mux/145
  Convert146/1 -> debug_mvdc_actuator_debug_T_max_Nm/1
  BusOutput/146 -> Convert146/1  "<T_max_Nm>"
  debug_mvdc_actuator_debug_T_max_Nm/1 -> Mux/146
  Convert147/1 -> debug_mvdc_actuator_debug_T_min_Nm/1
  BusOutput/147 -> Convert147/1  "<T_min_Nm>"
  debug_mvdc_actuator_debug_T_min_Nm/1 -> Mux/147
  Convert148/1 -> debug_mvdc_actuator_debug_T_engine_Nm/1
  BusOutput/148 -> Convert148/1  "<T_engine_Nm>"
  debug_mvdc_actuator_debug_T_engine_Nm/1 -> Mux/148
  Convert149/1 -> debug_mvdc_actuator_debug_p_Brake_bar/1
  BusOutput/149 -> Convert149/1  "<p_Brake_bar>"
  debug_mvdc_actuator_debug_p_Brake_bar/1 -> Mux/149
  Convert150/1 -> debug_mvdc_actuator_debug_p_throttle_pos/1
  BusOutput/150 -> Convert150/1  "<p_throttle_pos>"
  debug_mvdc_actuator_debug_p_throttle_pos/1 -> Mux/150
  Convert151/1 -> debug_mvdc_actuator_debug_gear/1
  BusOutput/151 -> Convert151/1  "<gear>"
  debug_mvdc_actuator_debug_gear/1 -> Mux/151
  Convert152/1 -> debug_ExternalDebug_UnixTime_s/1
  BusOutput/152 -> Convert152/1  "<UnixTime_s>"
  debug_ExternalDebug_UnixTime_s/1 -> Mux/152
  Convert153/1 -> debug_ExternalDebug_ExecutionTime_s/1
  BusOutput/153 -> Convert153/1  "<ExecutionTime_s>"
  debug_ExternalDebug_ExecutionTime_s/1 -> Mux/153
  Convert154/1 -> debug_ExternalDebug_ControlTime_s/1
  BusOutput/154 -> Convert154/1  "<ControlTime_s>"
  debug_ExternalDebug_ControlTime_s/1 -> Mux/154
  Convert155/1 -> debug_ExternalDebug_UpdateFrequency_Hz/1
  BusOutput/155 -> Convert155/1  "<UpdateFrequency_Hz>"
  debug_ExternalDebug_UpdateFrequency_Hz/1 -> Mux/155
  Convert156/1 -> debug_ExternalDebug_LostHeartbeatTimeout_s/1
  BusOutput/156 -> Convert156/1  "<LostHeartbeatTimeout_s>"
  debug_ExternalDebug_LostHeartbeatTimeout_s/1 -> Mux/156
  Convert157/1 -> debug_ExternalDebug_LostRaceControlTimeout_s/1
  BusOutput/157 -> Convert157/1  "<LostRaceControlTimeout_s>"
  debug_ExternalDebug_LostRaceControlTimeout_s/1 -> Mux/157
  Convert158/1 -> debug_ExternalDebug_DiagSD/1
  BusOutput/158 -> Convert158/1  "<DiagSD>"
  debug_ExternalDebug_DiagSD/1 -> Mux/158
  Convert159/1 -> debug_ExternalDebug_DiagMotec/1
  BusOutput/159 -> Convert159/1  "<DiagMotec>"
  debug_ExternalDebug_DiagMotec/1 -> Mux/159
  Convert160/1 -> debug_ExternalDebug_DiagOther/1
  BusOutput/160 -> Convert160/1  "<DiagOther>"
  debug_ExternalDebug_DiagOther/1 -> Mux/160
  Convert161/1 -> debug_mvdc_state_estimation_debug_StateEstimate_SE_Status/1
  BusOutput/161 -> Convert161/1  "<SE_Status>"
  debug_mvdc_state_estimation_debug_StateEstimate_SE_Status/1 -> Mux/161
  Convert162/1 -> debug_mvdc_state_estimation_debug_StateEstimate_SE_State/1
  BusOutput/162 -> Convert162/1  "<SE_State>"
  debug_mvdc_state_estimation_debug_StateEstimate_SE_State/1 -> Mux/162
  Convert163/1 -> debug_mvdc_state_estimation_debug_StateEstimate_Pos_x_m/1
  BusOutput/163 -> Convert163/1  "<x_m>"
  debug_mvdc_state_estimation_debug_StateEstimate_Pos_x_m/1 -> Mux/163
  Convert164/1 -> debug_mvdc_state_estimation_debug_StateEstimate_Pos_y_m/1
  BusOutput/164 -> Convert164/1  "<y_m>"
  debug_mvdc_state_estimation_debug_StateEstimate_Pos_y_m/1 -> Mux/164
  Convert165/1 -> debug_mvdc_state_estimation_debug_StateEstimate_Pos_psi_rad/1
  BusOutput/165 -> Convert165/1  "<psi_rad>"
  debug_mvdc_state_estimation_debug_StateEstimate_Pos_psi_rad/1 -> Mux/165
  Convert166/1 -> debug_mvdc_state_estimation_debug_StateEstimate_z_m/1
  BusOutput/166 -> Convert166/1  "<z_m>"
  debug_mvdc_state_estimation_debug_StateEstimate_z_m/1 -> Mux/166
  Convert167/1 -> debug_mvdc_state_estimation_debug_StateEstimate_PosAccuracy/1
  BusOutput/167 -> Convert167/1  "<PosAccuracy>"
  debug_mvdc_state_estimation_debug_StateEstimate_PosAccuracy/1 -> Mux/167
  Convert168/1 -> debug_mvdc_state_estimation_debug_StateEstimate_VelAccuracy/1
  BusOutput/168 -> Convert168/1  "<VelAccuracy>"
  debug_mvdc_state_estimation_debug_StateEstimate_VelAccuracy/1 -> Mux/168
  Convert169/1 -> debug_mvdc_state_estimation_debug_StateEstimate_dPsi_radps/1
  BusOutput/169 -> Convert169/1  "<dPsi_radps>"
  debug_mvdc_state_estimation_debug_StateEstimate_dPsi_radps/1 -> Mux/169
  Convert170/1 -> debug_mvdc_state_estimation_debug_StateEstimate_vx_mps/1
  BusOutput/170 -> Convert170/1  "<vx_mps>"
  debug_mvdc_state_estimation_debug_StateEstimate_vx_mps/1 -> Mux/170
  Convert171/1 -> debug_mvdc_state_estimation_debug_StateEstimate_vy_mps/1
  BusOutput/171 -> Convert171/1  "<vy_mps>"
  debug_mvdc_state_estimation_debug_StateEstimate_vy_mps/1 -> Mux/171
  Convert172/1 -> debug_mvdc_state_estimation_debug_StateEstimate_v_mps/1
  BusOutput/172 -> Convert172/1  "<v_mps>"
  debug_mvdc_state_estimation_debug_StateEstimate_v_mps/1 -> Mux/172
  Convert173/1 -> debug_mvdc_state_estimation_debug_StateEstimate_beta_rad/1
  BusOutput/173 -> Convert173/1  "<beta_rad>"
  debug_mvdc_state_estimation_debug_StateEstimate_beta_rad/1 -> Mux/173
  Convert174/1 -> debug_mvdc_state_estimation_debug_StateEstimate_ax_mps2/1
  BusOutput/174 -> Convert174/1  "<ax_mps2>"
  debug_mvdc_state_estimation_debug_StateEstimate_ax_mps2/1 -> Mux/174
  Convert175/1 -> debug_mvdc_state_estimation_debug_StateEstimate_ay_mps2/1
  BusOutput/175 -> Convert175/1  "<ay_mps2>"
  debug_mvdc_state_estimation_debug_StateEstimate_ay_mps2/1 -> Mux/175
  Convert176/1 -> debug_mvdc_state_estimation_debug_StateEstimate_valid_IMU_b/1
  BusOutput/176 -> Convert176/1  "<valid_IMU_b>"
  debug_mvdc_state_estimation_debug_StateEstimate_valid_IMU_b/1 -> Mux/176
  Convert177/1 -> debug_mvdc_state_estimation_debug_StateEstimate_psi_vel_rad/1
  BusOutput/177 -> Convert177/1  "<psi_vel_rad>"
  debug_mvdc_state_estimation_debug_StateEstimate_psi_vel_rad/1 -> Mux/177
  Convert178/1 -> debug_mvdc_state_estimation_debug_StateEstimate_kappa_radpm/1
  BusOutput/178 -> Convert178/1  "<kappa_radpm>"
  debug_mvdc_state_estimation_debug_StateEstimate_kappa_radpm/1 -> Mux/178
  Convert179/1 -> debug_mvdc_state_estimation_debug_StateEstimate_dBeta_radps/1
  BusOutput/179 -> Convert179/1  "<dBeta_radps>"
  debug_mvdc_state_estimation_debug_StateEstimate_dBeta_radps/1 -> Mux/179
  Convert180/1 -> debug_mvdc_state_estimation_debug_StateEstimate_ddPsi_radps2/1
  BusOutput/180 -> Convert180/1  "<ddPsi_radps2>"
  debug_mvdc_state_estimation_debug_StateEstimate_ddPsi_radps2/1 -> Mux/180
  Convert181/1 -> debug_mvdc_state_estimation_debug_StateEstimate_ax_vel_mps2/1
  BusOutput/181 -> Convert181/1  "<ax_vel_mps2>"
  debug_mvdc_state_estimation_debug_StateEstimate_ax_vel_mps2/1 -> Mux/181
  Convert182/1 -> debug_mvdc_state_estimation_debug_StateEstimate_ay_vel_mps2/1
  BusOutput/182 -> Convert182/1  "<ay_vel_mps2>"
  debug_mvdc_state_estimation_debug_StateEstimate_ay_vel_mps2/1 -> Mux/182
  Convert183/1 -> debug_mvdc_state_estimation_debug_StateEstimate_lambdaFL_perc/1
  BusOutput/183 -> Convert183/1  "<lambdaFL_perc>"
  debug_mvdc_state_estimation_debug_StateEstimate_lambdaFL_perc/1 -> Mux/183
  Convert184/1 -> debug_mvdc_state_estimation_debug_StateEstimate_lambdaFR_perc/1
  BusOutput/184 -> Convert184/1  "<lambdaFR_perc>"
  debug_mvdc_state_estimation_debug_StateEstimate_lambdaFR_perc/1 -> Mux/184
  Convert185/1 -> debug_mvdc_state_estimation_debug_StateEstimate_lambdaRL_perc/1
  BusOutput/185 -> Convert185/1  "<lambdaRL_perc>"
  debug_mvdc_state_estimation_debug_StateEstimate_lambdaRL_perc/1 -> Mux/185
  Convert186/1 -> debug_mvdc_state_estimation_debug_StateEstimate_lambdaRR_perc/1
  BusOutput/186 -> Convert186/1  "<lambdaRR_perc>"
  debug_mvdc_state_estimation_debug_StateEstimate_lambdaRR_perc/1 -> Mux/186
  Convert187/1 -> debug_mvdc_state_estimation_debug_StateEstimate_valid_Wheelspeeds_b/1
  BusOutput/187 -> Convert187/1  "<valid_Wheelspeeds_b>"
  debug_mvdc_state_estimation_debug_StateEstimate_valid_Wheelspeeds_b/1 -> Mux/187
  Convert188/1 -> debug_mvdc_state_estimation_debug_StateEstimate_alphaFL_rad/1
  BusOutput/188 -> Convert188/1  "<alphaFL_rad>"
  debug_mvdc_state_estimation_debug_StateEstimate_alphaFL_rad/1 -> Mux/188
  Convert189/1 -> debug_mvdc_state_estimation_debug_StateEstimate_alphaFR_rad/1
  BusOutput/189 -> Convert189/1  "<alphaFR_rad>"
  debug_mvdc_state_estimation_debug_StateEstimate_alphaFR_rad/1 -> Mux/189
  Convert190/1 -> debug_mvdc_state_estimation_debug_StateEstimate_alphaRL_rad/1
  BusOutput/190 -> Convert190/1  "<alphaRL_rad>"
  debug_mvdc_state_estimation_debug_StateEstimate_alphaRL_rad/1 -> Mux/190
  Convert191/1 -> debug_mvdc_state_estimation_debug_StateEstimate_alphaRR_rad/1
  BusOutput/191 -> Convert191/1  "<alphaRR_rad>"
  debug_mvdc_state_estimation_debug_StateEstimate_alphaRR_rad/1 -> Mux/191
  Convert192/1 -> debug_mvdc_state_estimation_debug_StateEstimate_DiffFRAlpha_rad/1
  BusOutput/192 -> Convert192/1  "<DiffFRAlpha_rad>"
  debug_mvdc_state_estimation_debug_StateEstimate_DiffFRAlpha_rad/1 -> Mux/192
  Convert193/1 -> debug_mvdc_state_estimation_debug_StateEstimate_DeltaWheel_rad/1
  BusOutput/193 -> Convert193/1  "<DeltaWheel_rad>"
  debug_mvdc_state_estimation_debug_StateEstimate_DeltaWheel_rad/1 -> Mux/193
  Convert194/1 -> debug_mvdc_state_estimation_debug_Residuals_res_xLoc1_m/1
  BusOutput/194 -> Convert194/1  "<res_xLoc1_m>"
  debug_mvdc_state_estimation_debug_Residuals_res_xLoc1_m/1 -> Mux/194
  Convert195/1 -> debug_mvdc_state_estimation_debug_Residuals_res_yLoc1_m/1
  BusOutput/195 -> Convert195/1  "<res_yLoc1_m>"
  debug_mvdc_state_estimation_debug_Residuals_res_yLoc1_m/1 -> Mux/195
  Convert196/1 -> debug_mvdc_state_estimation_debug_Residuals_res_psiLoc1_rad/1
  BusOutput/196 -> Convert196/1  "<res_psiLoc1_rad>"
  debug_mvdc_state_estimation_debug_Residuals_res_psiLoc1_rad/1 -> Mux/196
  Convert197/1 -> debug_mvdc_state_estimation_debug_Residuals_res_xLoc2_m/1
  BusOutput/197 -> Convert197/1  "<res_xLoc2_m>"
  debug_mvdc_state_estimation_debug_Residuals_res_xLoc2_m/1 -> Mux/197
  Convert198/1 -> debug_mvdc_state_estimation_debug_Residuals_res_yLoc2_m/1
  BusOutput/198 -> Convert198/1  "<res_yLoc2_m>"
  debug_mvdc_state_estimation_debug_Residuals_res_yLoc2_m/1 -> Mux/198
  Convert199/1 -> debug_mvdc_state_estimation_debug_Residuals_res_psiLoc2_rad/1
  BusOutput/199 -> Convert199/1  "<res_psiLoc2_rad>"
  debug_mvdc_state_estimation_debug_Residuals_res_psiLoc2_rad/1 -> Mux/199
  Convert200/1 -> debug_mvdc_state_estimation_debug_Residuals_res_xLoc3_m/1
  BusOutput/200 -> Convert200/1  "<res_xLoc3_m>"
  debug_mvdc_state_estimation_debug_Residuals_res_xLoc3_m/1 -> Mux/200
  Convert201/1 -> debug_mvdc_state_estimation_debug_Residuals_res_yLoc3_m/1
  BusOutput/201 -> Convert201/1  "<res_yLoc3_m>"
  debug_mvdc_state_estimation_debug_Residuals_res_yLoc3_m/1 -> Mux/201
  Convert202/1 -> debug_mvdc_state_estimation_debug_Residuals_res_psiLoc3_rad/1
  BusOutput/202 -> Convert202/1  "<res_psiLoc3_rad>"
  debug_mvdc_state_estimation_debug_Residuals_res_psiLoc3_rad/1 -> Mux/202
  Convert203/1 -> debug_mvdc_state_estimation_debug_Residuals_res_vxVel1_mps/1
  BusOutput/203 -> Convert203/1  "<res_vxVel1_mps>"
  debug_mvdc_state_estimation_debug_Residuals_res_vxVel1_mps/1 -> Mux/203
  Convert204/1 -> debug_mvdc_state_estimation_debug_Residuals_res_vyVel1_mps/1
  BusOutput/204 -> Convert204/1  "<res_vyVel1_mps>"
  debug_mvdc_state_estimation_debug_Residuals_res_vyVel1_mps/1 -> Mux/204
  Convert205/1 -> debug_mvdc_state_estimation_debug_Residuals_res_vxVel2_mps/1
  BusOutput/205 -> Convert205/1  "<res_vxVel2_mps>"
  debug_mvdc_state_estimation_debug_Residuals_res_vxVel2_mps/1 -> Mux/205
  Convert206/1 -> debug_mvdc_state_estimation_debug_Residuals_res_vyVel2_mps/1
  BusOutput/206 -> Convert206/1  "<res_vyVel2_mps>"
  debug_mvdc_state_estimation_debug_Residuals_res_vyVel2_mps/1 -> Mux/206
  Convert207/1 -> debug_mvdc_state_estimation_debug_Residuals_res_dPsi1_radps/1
  BusOutput/207 -> Convert207/1  "<res_dPsi1_radps>"
  debug_mvdc_state_estimation_debug_Residuals_res_dPsi1_radps/1 -> Mux/207
  Convert208/1 -> debug_mvdc_state_estimation_debug_Residuals_res_dPsi2_radps/1
  BusOutput/208 -> Convert208/1  "<res_dPsi2_radps>"
  debug_mvdc_state_estimation_debug_Residuals_res_dPsi2_radps/1 -> Mux/208
  Convert209/1 -> debug_mvdc_state_estimation_debug_Residuals_res_sLoc1_m/1
  BusOutput/209 -> Convert209/1  "<res_sLoc1_m>"
  debug_mvdc_state_estimation_debug_Residuals_res_sLoc1_m/1 -> Mux/209
  Convert210/1 -> debug_mvdc_state_estimation_debug_Residuals_res_dLoc1_m/1
  BusOutput/210 -> Convert210/1  "<res_dLoc1_m>"
  debug_mvdc_state_estimation_debug_Residuals_res_dLoc1_m/1 -> Mux/210
  Convert211/1 -> debug_mvdc_state_estimation_debug_Residuals_res_sLoc2_m/1
  BusOutput/211 -> Convert211/1  "<res_sLoc2_m>"
  debug_mvdc_state_estimation_debug_Residuals_res_sLoc2_m/1 -> Mux/211
  Convert212/1 -> debug_mvdc_state_estimation_debug_Residuals_res_dLoc2_m/1
  BusOutput/212 -> Convert212/1  "<res_dLoc2_m>"
  debug_mvdc_state_estimation_debug_Residuals_res_dLoc2_m/1 -> Mux/212
  Convert213/1 -> debug_mvdc_state_estimation_debug_Residuals_res_sLoc3_m/1
  BusOutput/213 -> Convert213/1  "<res_sLoc3_m>"
  debug_mvdc_state_estimation_debug_Residuals_res_sLoc3_m/1 -> Mux/213
  Convert214/1 -> debug_mvdc_state_estimation_debug_Residuals_res_dLoc3_m/1
  BusOutput/214 -> Convert214/1  "<res_dLoc3_m>"
  debug_mvdc_state_estimation_debug_Residuals_res_dLoc3_m/1 -> Mux/214
  Convert215/1 -> debug_mvdc_state_estimation_debug_Diagnosis_valid_Loc1_b/1
  BusOutput/215 -> Convert215/1  "<valid_Loc1_b>"
  debug_mvdc_state_estimation_debug_Diagnosis_valid_Loc1_b/1 -> Mux/215
  Convert216/1 -> debug_mvdc_state_estimation_debug_Diagnosis_valid_Loc2_b/1
  BusOutput/216 -> Convert216/1  "<valid_Loc2_b>"
  debug_mvdc_state_estimation_debug_Diagnosis_valid_Loc2_b/1 -> Mux/216
  Convert217/1 -> debug_mvdc_state_estimation_debug_Diagnosis_valid_Loc3_b/1
  BusOutput/217 -> Convert217/1  "<valid_Loc3_b>"
  debug_mvdc_state_estimation_debug_Diagnosis_valid_Loc3_b/1 -> Mux/217
  Convert218/1 -> debug_mvdc_state_estimation_debug_Diagnosis_valid_Vel1_b/1
  BusOutput/218 -> Convert218/1  "<valid_Vel1_b>"
  debug_mvdc_state_estimation_debug_Diagnosis_valid_Vel1_b/1 -> Mux/218
  Convert219/1 -> debug_mvdc_state_estimation_debug_Diagnosis_valid_Vel2_b/1
  BusOutput/219 -> Convert219/1  "<valid_Vel2_b>"
  debug_mvdc_state_estimation_debug_Diagnosis_valid_Vel2_b/1 -> Mux/219
  Convert220/1 -> debug_mvdc_state_estimation_debug_Diagnosis_valid_IMU1_b/1
  BusOutput/220 -> Convert220/1  "<valid_IMU1_b>"
  debug_mvdc_state_estimation_debug_Diagnosis_valid_IMU1_b/1 -> Mux/220
  Convert221/1 -> debug_mvdc_state_estimation_debug_Diagnosis_valid_IMU2_b/1
  BusOutput/221 -> Convert221/1  "<valid_IMU2_b>"
  debug_mvdc_state_estimation_debug_Diagnosis_valid_IMU2_b/1 -> Mux/221
  Convert222/1 -> debug_mvdc_state_estimation_debug_Diagnosis_fail_Loc1_b/1
  BusOutput/222 -> Convert222/1  "<fail_Loc1_b>"
  debug_mvdc_state_estimation_debug_Diagnosis_fail_Loc1_b/1 -> Mux/222
  Convert223/1 -> debug_mvdc_state_estimation_debug_Diagnosis_fail_Loc2_b/1
  BusOutput/223 -> Convert223/1  "<fail_Loc2_b>"
  debug_mvdc_state_estimation_debug_Diagnosis_fail_Loc2_b/1 -> Mux/223
  Convert224/1 -> debug_mvdc_state_estimation_debug_Diagnosis_fail_Loc3_b/1
  BusOutput/224 -> Convert224/1  "<fail_Loc3_b>"
  debug_mvdc_state_estimation_debug_Diagnosis_fail_Loc3_b/1 -> Mux/224
  Convert225/1 -> debug_mvdc_state_estimation_debug_Diagnosis_fail_Vel1_b/1
  BusOutput/225 -> Convert225/1  "<fail_Vel1_b>"
  debug_mvdc_state_estimation_debug_Diagnosis_fail_Vel1_b/1 -> Mux/225
  Convert226/1 -> debug_mvdc_state_estimation_debug_Diagnosis_fail_Vel2_b/1
  BusOutput/226 -> Convert226/1  "<fail_Vel2_b>"
  debug_mvdc_state_estimation_debug_Diagnosis_fail_Vel2_b/1 -> Mux/226
  Convert227/1 -> debug_mvdc_state_estimation_debug_Diagnosis_fail_IMU1_b/1
  BusOutput/227 -> Convert227/1  "<fail_IMU1_b>"
  debug_mvdc_state_estimation_debug_Diagnosis_fail_IMU1_b/1 -> Mux/227
  Convert228/1 -> debug_mvdc_state_estimation_debug_Diagnosis_fail_IMU2_b/1
  BusOutput/228 -> Convert228/1  "<fail_IMU2_b>"
  debug_mvdc_state_estimation_debug_Diagnosis_fail_IMU2_b/1 -> Mux/228
  Convert229/1 -> debug_mvdc_state_estimation_debug_Odom_Position_x_m/1
  BusOutput/229 -> Convert229/1  "<x_m>"
  debug_mvdc_state_estimation_debug_Odom_Position_x_m/1 -> Mux/229
  Convert230/1 -> debug_mvdc_state_estimation_debug_Odom_Position_y_m/1
  BusOutput/230 -> Convert230/1  "<y_m>"
  debug_mvdc_state_estimation_debug_Odom_Position_y_m/1 -> Mux/230
  Convert231/1 -> debug_mvdc_state_estimation_debug_Odom_Position_psi_rad/1
  BusOutput/231 -> Convert231/1  "<psi_rad>"
  debug_mvdc_state_estimation_debug_Odom_Position_psi_rad/1 -> Mux/231
  Convert232/1 -> debug_mvdc_state_estimation_debug_Odom_Valid_b/1
  BusOutput/232 -> Convert232/1  "<Valid_b>"
  debug_mvdc_state_estimation_debug_Odom_Valid_b/1 -> Mux/232
  Convert233/1 -> debug_mloc_statemachine_debug_Hardware_Status/1
  BusOutput/233 -> Convert233/1  "<Hardware_Status>"
  debug_mloc_statemachine_debug_Hardware_Status/1 -> Mux/233
  Convert234/1 -> debug_mloc_statemachine_debug_AIDriver_Status/1
  BusOutput/234 -> Convert234/1  "<AIDriver_Status>"
  debug_mloc_statemachine_debug_AIDriver_Status/1 -> Mux/234
  Convert235/1 -> debug_mloc_statemachine_debug_ParkBrakeApplied_b/1
  BusOutput/235 -> Convert235/1  "<ParkBrakeApplied_b>"
  debug_mloc_statemachine_debug_ParkBrakeApplied_b/1 -> Mux/235
  Convert236/1 -> debug_mloc_statemachine_debug_VehicleReady2Drive/1
  BusOutput/236 -> Convert236/1  "<VehicleReady2Drive>"
  debug_mloc_statemachine_debug_VehicleReady2Drive/1 -> Mux/236
  Convert237/1 -> debug_mloc_statemachine_debug_StateEstimation_Status/1
  BusOutput/237 -> Convert237/1  "<StateEstimation_Status>"
  debug_mloc_statemachine_debug_StateEstimation_Status/1 -> Mux/237
  Convert238/1 -> debug_mloc_statemachine_debug_VehicleSafeStandstill/1
  BusOutput/238 -> Convert238/1  "<VehicleSafeStandstill>"
  debug_mloc_statemachine_debug_VehicleSafeStandstill/1 -> Mux/238
  Convert239/1 -> debug_mloc_statemachine_debug_Driver_Status/1
  BusOutput/239 -> Convert239/1  "<Driver_Status>"
  debug_mloc_statemachine_debug_Driver_Status/1 -> Mux/239
  Convert240/1 -> debug_mloc_statemachine_debug_VehicleUnsafe/1
  BusOutput/240 -> Convert240/1  "<VehicleUnsafe>"
  debug_mloc_statemachine_debug_VehicleUnsafe/1 -> Mux/240
  Convert241/1 -> debug_mloc_statemachine_debug_TUMVehicleState/1
  BusOutput/241 -> Convert241/1  "<TUMVehicleState>"
  debug_mloc_statemachine_debug_TUMVehicleState/1 -> Mux/241
  Convert242/1 -> debug_mloc_statemachine_debug_EnableSensorFusion/1
  BusOutput/242 -> Convert242/1  "<EnableSensorFusion>"
  debug_mloc_statemachine_debug_EnableSensorFusion/1 -> Mux/242
  Convert243/1 -> debug_mloc_statemachine_debug_EnableControlOutputs/1
  BusOutput/243 -> Convert243/1  "<EnableControlOutputs>"
  debug_mloc_statemachine_debug_EnableControlOutputs/1 -> Mux/243
  Convert244/1 -> debug_mloc_statemachine_debug_EnableDriver/1
  BusOutput/244 -> Convert244/1  "<EnableDriver>"
  debug_mloc_statemachine_debug_EnableDriver/1 -> Mux/244
  Convert245/1 -> debug_mloc_statemachine_debug_EnableHardEmergencyBrake/1
  BusOutput/245 -> Convert245/1  "<EnableHardEmergencyBrake>"
  debug_mloc_statemachine_debug_EnableHardEmergencyBrake/1 -> Mux/245
  Convert246/1 -> debug_mloc_statemachine_debug_RequestControl/1
  BusOutput/246 -> Convert246/1  "<RequestControl>"
  debug_mloc_statemachine_debug_RequestControl/1 -> Mux/246
  Convert247/1 -> debug_VehicleSensorData_s_DamperPotsFL_mm/1
  BusOutput/247 -> Convert247/1  "<s_DamperPotsFL_mm>"
  debug_VehicleSensorData_s_DamperPotsFL_mm/1 -> Mux/247
  Convert248/1 -> debug_VehicleSensorData_s_DamperPotsFR_mm/1
  BusOutput/248 -> Convert248/1  "<s_DamperPotsFR_mm>"
  debug_VehicleSensorData_s_DamperPotsFR_mm/1 -> Mux/248
  Convert249/1 -> debug_VehicleSensorData_s_DamperPotsRL_mm/1
  BusOutput/249 -> Convert249/1  "<s_DamperPotsRL_mm>"
  debug_VehicleSensorData_s_DamperPotsRL_mm/1 -> Mux/249
  Convert250/1 -> debug_VehicleSensorData_s_DamperPotsRR_mm/1
  BusOutput/250 -> Convert250/1  "<s_DamperPotsRR_mm>"
  debug_VehicleSensorData_s_DamperPotsRR_mm/1 -> Mux/250
  Convert251/1 -> debug_VehicleSensorData_p_TirePressureFL_bar/1
  BusOutput/251 -> Convert251/1  "<p_TirePressureFL_bar>"
  debug_VehicleSensorData_p_TirePressureFL_bar/1 -> Mux/251
  Convert252/1 -> debug_VehicleSensorData_p_TirePressureFR_bar/1
  BusOutput/252 -> Convert252/1  "<p_TirePressureFR_bar>"
  debug_VehicleSensorData_p_TirePressureFR_bar/1 -> Mux/252
  Convert253/1 -> debug_VehicleSensorData_p_TirePressureRL_bar/1
  BusOutput/253 -> Convert253/1  "<p_TirePressureRL_bar>"
  debug_VehicleSensorData_p_TirePressureRL_bar/1 -> Mux/253
  Convert254/1 -> debug_VehicleSensorData_p_TirePressureRR_bar/1
  BusOutput/254 -> Convert254/1  "<p_TirePressureRR_bar>"
  debug_VehicleSensorData_p_TirePressureRR_bar/1 -> Mux/254
  Convert255/1 -> debug_VehicleSensorData_T_TireFL_Celsius/1
  BusOutput/255 -> Convert255/1  "<T_TireFL_Celsius>"
  debug_VehicleSensorData_T_TireFL_Celsius/1 -> Mux/255
  Convert256/1 -> debug_VehicleSensorData_T_TireFR_Celsius/1
  BusOutput/256 -> Convert256/1  "<T_TireFR_Celsius>"
  debug_VehicleSensorData_T_TireFR_Celsius/1 -> Mux/256
  Convert257/1 -> debug_VehicleSensorData_T_TireRL_Celsius/1
  BusOutput/257 -> Convert257/1  "<T_TireRL_Celsius>"
  debug_VehicleSensorData_T_TireRL_Celsius/1 -> Mux/257
  Convert258/1 -> debug_VehicleSensorData_T_TireRR_Celsius/1
  BusOutput/258 -> Convert258/1  "<T_TireRR_Celsius>"
  debug_VehicleSensorData_T_TireRR_Celsius/1 -> Mux/258
  Convert259/1 -> debug_VehicleSensorData_BatteryVoltage_V/1
  BusOutput/259 -> Convert259/1  "<BatteryVoltage_V>"
  debug_VehicleSensorData_BatteryVoltage_V/1 -> Mux/259
  Convert260/1 -> debug_VehicleSensorData_Delta_Manual_rad/1
  BusOutput/260 -> Convert260/1  "<Delta_Manual_rad>"
  debug_VehicleSensorData_Delta_Manual_rad/1 -> Mux/260
  Convert261/1 -> debug_VehicleSensorData_Throttle_Manual_perc/1
  BusOutput/261 -> Convert261/1  "<Throttle_Manual_perc>"
  debug_VehicleSensorData_Throttle_Manual_perc/1 -> Mux/261
  Convert262/1 -> debug_VehicleSensorData_Brake_Manual_bar/1
  BusOutput/262 -> Convert262/1  "<Brake_Manual_bar>"
  debug_VehicleSensorData_Brake_Manual_bar/1 -> Mux/262
  Convert263/1 -> debug_VehicleSensorData_Gear_Manual/1
  BusOutput/263 -> Convert263/1  "<Gear_Manual>"
  debug_VehicleSensorData_Gear_Manual/1 -> Mux/263
  Convert264/1 -> debug_VehicleSensorData_T_CoolantTemp_Celsius/1
  BusOutput/264 -> Convert264/1  "<T_CoolantTemp_Celsius>"
  debug_VehicleSensorData_T_CoolantTemp_Celsius/1 -> Mux/264
  Convert265/1 -> debug_VehicleSensorData_T_TransmissionOilTemp_Celsius/1
  BusOutput/265 -> Convert265/1  "<T_TransmissionOilTemp_Celsius>"
  debug_VehicleSensorData_T_TransmissionOilTemp_Celsius/1 -> Mux/265
  Convert266/1 -> debug_VehicleSensorData_p_Fuel_kPa/1
  BusOutput/266 -> Convert266/1  "<p_Fuel_kPa>"
  debug_VehicleSensorData_p_Fuel_kPa/1 -> Mux/266
  Convert267/1 -> debug_VehicleSensorData_p_EngineOil_kPa/1
  BusOutput/267 -> Convert267/1  "<p_EngineOil_kPa>"
  debug_VehicleSensorData_p_EngineOil_kPa/1 -> Mux/267
  Convert268/1 -> debug_VehicleSensorData_Tz_Powertrain_Nm/1
  BusOutput/268 -> Convert268/1  "<Tz_Powertrain_Nm>"
  debug_VehicleSensorData_Tz_Powertrain_Nm/1 -> Mux/268
  Convert269/1 -> debug_VehicleSensorData_T_Engine_Nm/1
  BusOutput/269 -> Convert269/1  "<T_Engine_Nm>"
  debug_VehicleSensorData_T_Engine_Nm/1 -> Mux/269
  Convert270/1 -> debug_VehicleSensorData_GearEngaged/1
  BusOutput/270 -> Convert270/1  "<GearEngaged>"
  debug_VehicleSensorData_GearEngaged/1 -> Mux/270
  Convert271/1 -> debug_VehicleSensorData_omega_Engine_radps/1
  BusOutput/271 -> Convert271/1  "<omega_Engine_radps>"
  debug_VehicleSensorData_omega_Engine_radps/1 -> Mux/271
  Convert272/1 -> debug_VehicleSensorData_ThrottlePos_perc/1
  BusOutput/272 -> Convert272/1  "<ThrottlePos_perc>"
  debug_VehicleSensorData_ThrottlePos_perc/1 -> Mux/272
  Convert273/1 -> debug_VehicleSensorData_T_WheelFL_Nm/1
  BusOutput/273 -> Convert273/1  "<T_WheelFL_Nm>"
  debug_VehicleSensorData_T_WheelFL_Nm/1 -> Mux/273
  Convert274/1 -> debug_VehicleSensorData_T_WheelFR_Nm/1
  BusOutput/274 -> Convert274/1  "<T_WheelFR_Nm>"
  debug_VehicleSensorData_T_WheelFR_Nm/1 -> Mux/274
  Convert275/1 -> debug_VehicleSensorData_T_WheelRL_Nm/1
  BusOutput/275 -> Convert275/1  "<T_WheelRL_Nm>"
  debug_VehicleSensorData_T_WheelRL_Nm/1 -> Mux/275
  Convert276/1 -> debug_VehicleSensorData_T_WheelRR_Nm/1
  BusOutput/276 -> Convert276/1  "<T_WheelRR_Nm>"
  debug_VehicleSensorData_T_WheelRR_Nm/1 -> Mux/276
  Convert277/1 -> debug_VehicleSensorData_Delta_Wheel_rad/1
  BusOutput/277 -> Convert277/1  "<Delta_Wheel_rad>"
  debug_VehicleSensorData_Delta_Wheel_rad/1 -> Mux/277
  Convert278/1 -> debug_VehicleSensorData_p_BrakeF_bar/1
  BusOutput/278 -> Convert278/1  "<p_BrakeF_bar>"
  debug_VehicleSensorData_p_BrakeF_bar/1 -> Mux/278
  Convert279/1 -> debug_VehicleSensorData_p_BrakeR_bar/1
  BusOutput/279 -> Convert279/1  "<p_BrakeR_bar>"
  debug_VehicleSensorData_p_BrakeR_bar/1 -> Mux/279
  Convert280/1 -> debug_VehicleSensorData_omega_WheelFL_radps/1
  BusOutput/280 -> Convert280/1  "<omega_WheelFL_radps>"
  debug_VehicleSensorData_omega_WheelFL_radps/1 -> Mux/280
  Convert281/1 -> debug_VehicleSensorData_omega_WheelFR_radps/1
  BusOutput/281 -> Convert281/1  "<omega_WheelFR_radps>"
  debug_VehicleSensorData_omega_WheelFR_radps/1 -> Mux/281
  Convert282/1 -> debug_VehicleSensorData_omega_WheelRL_radps/1
  BusOutput/282 -> Convert282/1  "<omega_WheelRL_radps>"
  debug_VehicleSensorData_omega_WheelRL_radps/1 -> Mux/282
  Convert283/1 -> debug_VehicleSensorData_omega_WheelRR_radps/1
  BusOutput/283 -> Convert283/1  "<omega_WheelRR_radps>"
  debug_VehicleSensorData_omega_WheelRR_radps/1 -> Mux/283
  Convert284/1 -> debug_VehicleSensorData_valid_Wheelspeeds_b/1
  BusOutput/284 -> Convert284/1  "<valid_Wheelspeeds_b>"
  debug_VehicleSensorData_valid_Wheelspeeds_b/1 -> Mux/284
  Convert285/1 -> debug_VehicleSensorData_x_Loc1_m/1
  BusOutput/285 -> Convert285/1  "<x_Loc1_m>"
  debug_VehicleSensorData_x_Loc1_m/1 -> Mux/285
  Convert286/1 -> debug_VehicleSensorData_y_Loc1_m/1
  BusOutput/286 -> Convert286/1  "<y_Loc1_m>"
  debug_VehicleSensorData_y_Loc1_m/1 -> Mux/286
  Convert287/1 -> debug_VehicleSensorData_z_Loc1_m/1
  BusOutput/287 -> Convert287/1  "<z_Loc1_m>"
  debug_VehicleSensorData_z_Loc1_m/1 -> Mux/287
  Convert288/1 -> debug_VehicleSensorData_phi_RollAngleLoc1_rad/1
  BusOutput/288 -> Convert288/1  "<phi_RollAngleLoc1_rad>"
  debug_VehicleSensorData_phi_RollAngleLoc1_rad/1 -> Mux/288
  Convert289/1 -> debug_VehicleSensorData_theta_PitchAngleLoc1_rad/1
  BusOutput/289 -> Convert289/1  "<theta_PitchAngleLoc1_rad>"
  debug_VehicleSensorData_theta_PitchAngleLoc1_rad/1 -> Mux/289
  Convert290/1 -> debug_VehicleSensorData_psi_YawAngleLoc1_rad/1
  BusOutput/290 -> Convert290/1  "<psi_YawAngleLoc1_rad>"
  debug_VehicleSensorData_psi_YawAngleLoc1_rad/1 -> Mux/290
  Convert291/1 -> debug_VehicleSensorData_t_EstimateLoc1_s/1
  BusOutput/291 -> Convert291/1  "<t_EstimateLoc1_s>"
  debug_VehicleSensorData_t_EstimateLoc1_s/1 -> Mux/291
  Convert292/1 -> debug_VehicleSensorData_valid_Loc1_b/1
  BusOutput/292 -> Convert292/1  "<valid_Loc1_b>"
  debug_VehicleSensorData_valid_Loc1_b/1 -> Mux/292
  Convert293/1 -> debug_VehicleSensorData_accuracy_Loc1/1
  BusOutput/293 -> Convert293/1  "<accuracy_Loc1>"
  debug_VehicleSensorData_accuracy_Loc1/1 -> Mux/293
  Convert294/1 -> debug_VehicleSensorData_x_Loc2_m/1
  BusOutput/294 -> Convert294/1  "<x_Loc2_m>"
  debug_VehicleSensorData_x_Loc2_m/1 -> Mux/294
  Convert295/1 -> debug_VehicleSensorData_y_Loc2_m/1
  BusOutput/295 -> Convert295/1  "<y_Loc2_m>"
  debug_VehicleSensorData_y_Loc2_m/1 -> Mux/295
  Convert296/1 -> debug_VehicleSensorData_z_Loc2_m/1
  BusOutput/296 -> Convert296/1  "<z_Loc2_m>"
  debug_VehicleSensorData_z_Loc2_m/1 -> Mux/296
  Convert297/1 -> debug_VehicleSensorData_phi_RollAngleLoc2_rad/1
  BusOutput/297 -> Convert297/1  "<phi_RollAngleLoc2_rad>"
  debug_VehicleSensorData_phi_RollAngleLoc2_rad/1 -> Mux/297
  Convert298/1 -> debug_VehicleSensorData_theta_PitchAngleLoc2_rad/1
  BusOutput/298 -> Convert298/1  "<theta_PitchAngleLoc2_rad>"
  debug_VehicleSensorData_theta_PitchAngleLoc2_rad/1 -> Mux/298
  Convert299/1 -> debug_VehicleSensorData_psi_YawAngleLoc2_rad/1
  BusOutput/299 -> Convert299/1  "<psi_YawAngleLoc2_rad>"
  debug_VehicleSensorData_psi_YawAngleLoc2_rad/1 -> Mux/299
  Convert300/1 -> debug_VehicleSensorData_t_EstimateLoc2_s/1
  BusOutput/300 -> Convert300/1  "<t_EstimateLoc2_s>"
  debug_VehicleSensorData_t_EstimateLoc2_s/1 -> Mux/300
  Convert301/1 -> debug_VehicleSensorData_valid_Loc2_b/1
  BusOutput/301 -> Convert301/1  "<valid_Loc2_b>"
  debug_VehicleSensorData_valid_Loc2_b/1 -> Mux/301
  Convert302/1 -> debug_VehicleSensorData_accuracy_Loc2/1
  BusOutput/302 -> Convert302/1  "<accuracy_Loc2>"
  debug_VehicleSensorData_accuracy_Loc2/1 -> Mux/302
  Convert303/1 -> debug_VehicleSensorData_x_Loc3_m/1
  BusOutput/303 -> Convert303/1  "<x_Loc3_m>"
  debug_VehicleSensorData_x_Loc3_m/1 -> Mux/303
  Convert304/1 -> debug_VehicleSensorData_y_Loc3_m/1
  BusOutput/304 -> Convert304/1  "<y_Loc3_m>"
  debug_VehicleSensorData_y_Loc3_m/1 -> Mux/304
  Convert305/1 -> debug_VehicleSensorData_z_Loc3_m/1
  BusOutput/305 -> Convert305/1  "<z_Loc3_m>"
  debug_VehicleSensorData_z_Loc3_m/1 -> Mux/305
  Convert306/1 -> debug_VehicleSensorData_phi_RollAngleLoc3_rad/1
  BusOutput/306 -> Convert306/1  "<phi_RollAngleLoc3_rad>"
  debug_VehicleSensorData_phi_RollAngleLoc3_rad/1 -> Mux/306
  Convert307/1 -> debug_VehicleSensorData_theta_PitchAngleLoc3_rad/1
  BusOutput/307 -> Convert307/1  "<theta_PitchAngleLoc3_rad>"
  debug_VehicleSensorData_theta_PitchAngleLoc3_rad/1 -> Mux/307
  Convert308/1 -> debug_VehicleSensorData_psi_YawAngleLoc3_rad/1
  BusOutput/308 -> Convert308/1  "<psi_YawAngleLoc3_rad>"
  debug_VehicleSensorData_psi_YawAngleLoc3_rad/1 -> Mux/308
  Convert309/1 -> debug_VehicleSensorData_t_EstimateLoc3_s/1
  BusOutput/309 -> Convert309/1  "<t_EstimateLoc3_s>"
  debug_VehicleSensorData_t_EstimateLoc3_s/1 -> Mux/309
  Convert310/1 -> debug_VehicleSensorData_valid_Loc3_b/1
  BusOutput/310 -> Convert310/1  "<valid_Loc3_b>"
  debug_VehicleSensorData_valid_Loc3_b/1 -> Mux/310
  Convert311/1 -> debug_VehicleSensorData_accuracy_Loc3/1
  BusOutput/311 -> Convert311/1  "<accuracy_Loc3>"
  debug_VehicleSensorData_accuracy_Loc3/1 -> Mux/311
  Convert312/1 -> debug_VehicleSensorData_vx_CoGVel1_mps/1
  BusOutput/312 -> Convert312/1  "<vx_CoGVel1_mps>"
  debug_VehicleSensorData_vx_CoGVel1_mps/1 -> Mux/312
  Convert313/1 -> debug_VehicleSensorData_vy_CoGVel1_mps/1
  BusOutput/313 -> Convert313/1  "<vy_CoGVel1_mps>"
  debug_VehicleSensorData_vy_CoGVel1_mps/1 -> Mux/313
  Convert314/1 -> debug_VehicleSensorData_valid_Vel1_b/1
  BusOutput/314 -> Convert314/1  "<valid_Vel1_b>"
  debug_VehicleSensorData_valid_Vel1_b/1 -> Mux/314
  Convert315/1 -> debug_VehicleSensorData_vx_CoGVel2_mps/1
  BusOutput/315 -> Convert315/1  "<vx_CoGVel2_mps>"
  debug_VehicleSensorData_vx_CoGVel2_mps/1 -> Mux/315
  Convert316/1 -> debug_VehicleSensorData_vy_CoGVel2_mps/1
  BusOutput/316 -> Convert316/1  "<vy_CoGVel2_mps>"
  debug_VehicleSensorData_vy_CoGVel2_mps/1 -> Mux/316
  Convert317/1 -> debug_VehicleSensorData_valid_Vel2_b/1
  BusOutput/317 -> Convert317/1  "<valid_Vel2_b>"
  debug_VehicleSensorData_valid_Vel2_b/1 -> Mux/317
  Convert318/1 -> debug_VehicleSensorData_ax_CoGIMU1_mps2/1
  BusOutput/318 -> Convert318/1  "<ax_CoGIMU1_mps2>"
  debug_VehicleSensorData_ax_CoGIMU1_mps2/1 -> Mux/318
  Convert319/1 -> debug_VehicleSensorData_ay_CoGIMU1_mps2/1
  BusOutput/319 -> Convert319/1  "<ay_CoGIMU1_mps2>"
  debug_VehicleSensorData_ay_CoGIMU1_mps2/1 -> Mux/319
  Convert320/1 -> debug_VehicleSensorData_az_CoGIMU1_mps2/1
  BusOutput/320 -> Convert320/1  "<az_CoGIMU1_mps2>"
  debug_VehicleSensorData_az_CoGIMU1_mps2/1 -> Mux/320
  Convert321/1 -> debug_VehicleSensorData_dPhi_RollRateIMU1_radps/1
  BusOutput/321 -> Convert321/1  "<dPhi_RollRateIMU1_radps>"
  debug_VehicleSensorData_dPhi_RollRateIMU1_radps/1 -> Mux/321
  Convert322/1 -> debug_VehicleSensorData_dTheta_PitchRateIMU1_radps/1
  BusOutput/322 -> Convert322/1  "<dTheta_PitchRateIMU1_radps>"
  debug_VehicleSensorData_dTheta_PitchRateIMU1_radps/1 -> Mux/322
  Convert323/1 -> debug_VehicleSensorData_dPsi_YawRateIMU1_radps/1
  BusOutput/323 -> Convert323/1  "<dPsi_YawRateIMU1_radps>"
  debug_VehicleSensorData_dPsi_YawRateIMU1_radps/1 -> Mux/323
  Convert324/1 -> debug_VehicleSensorData_valid_IMU1_b/1
  BusOutput/324 -> Convert324/1  "<valid_IMU1_b>"
  debug_VehicleSensorData_valid_IMU1_b/1 -> Mux/324
  Convert325/1 -> debug_VehicleSensorData_ax_CoGIMU2_mps2/1
  BusOutput/325 -> Convert325/1  "<ax_CoGIMU2_mps2>"
  debug_VehicleSensorData_ax_CoGIMU2_mps2/1 -> Mux/325
  Convert326/1 -> debug_VehicleSensorData_ay_CoGIMU2_mps2/1
  BusOutput/326 -> Convert326/1  "<ay_CoGIMU2_mps2>"
  debug_VehicleSensorData_ay_CoGIMU2_mps2/1 -> Mux/326
  Convert327/1 -> debug_VehicleSensorData_az_CoGIMU2_mps2/1
  BusOutput/327 -> Convert327/1  "<az_CoGIMU2_mps2>"
  debug_VehicleSensorData_az_CoGIMU2_mps2/1 -> Mux/327
  Convert328/1 -> debug_VehicleSensorData_dPhi_RollRateIMU2_radps/1
  BusOutput/328 -> Convert328/1  "<dPhi_RollRateIMU2_radps>"
  debug_VehicleSensorData_dPhi_RollRateIMU2_radps/1 -> Mux/328
  Convert329/1 -> debug_VehicleSensorData_dTheta_PitchRateIMU2_radps/1
  BusOutput/329 -> Convert329/1  "<dTheta_PitchRateIMU2_radps>"
  debug_VehicleSensorData_dTheta_PitchRateIMU2_radps/1 -> Mux/329
  Convert330/1 -> debug_VehicleSensorData_dPsi_YawRateIMU2_radps/1
  BusOutput/330 -> Convert330/1  "<dPsi_YawRateIMU2_radps>"
  debug_VehicleSensorData_dPsi_YawRateIMU2_radps/1 -> Mux/330
  Convert331/1 -> debug_VehicleSensorData_valid_IMU2_b/1
  BusOutput/331 -> Convert331/1  "<valid_IMU2_b>"
  debug_VehicleSensorData_valid_IMU2_b/1 -> Mux/331
  Convert332/1 -> debug_Time_s/1
  BusOutput/332 -> Convert332/1  "<Time_s>"
  debug_Time_s/1 -> Mux/332
  Mux/1 -> DebugOut/1
